simulink model "sim_tvt_2025_pos_ctrl"  (R2020a)
settings: Solver=ode4  StartTime=0.0  StopTime=30.0  FixedStep=0.01  RelTol=1e-3
values from neighbouring files (symbols this model uses):
  alfa = 0.02    [init_tvt_2025_pos_ctrl.m]
  alfa_theta = 20    [init_tvt_2025_pos_ctrl.m]
  alfa_theta_obs = 100    [init_tvt_2025_pos_ctrl.m]
  c0 = 0.1    [init_tvt_2025_pos_ctrl.m]
  c1_diff_sigma_bar_v = diag([25; 30; 20])    [init_tvt_2025_pos_ctrl.m]
  c1v = diag([5.8; 6.5; 6.5])    [init_tvt_2025_pos_ctrl.m]
  c2_diff_sigma_bar_v = diag([50; 50; 10])    [init_tvt_2025_pos_ctrl.m]
  c2v = diag([5.8; 6.5; 6.5])    [init_tvt_2025_pos_ctrl.m]
  c3_diff_sigma_bar_v = diag([15; 15; 10])    [init_tvt_2025_pos_ctrl.m]
  c3v = diag([4.8; 6.4; 6.0])    [init_tvt_2025_pos_ctrl.m]
  delta_p_i_0 = zeros(3, NF)    [init_tvt_2025_pos_ctrl.m]
  delta_v_i_0 = zeros(3, NF)    [init_tvt_2025_pos_ctrl.m]
  dp_aa_t = 0.2 * ones(3, 5) + ( 1.0 - 0.2 ) * rand(3, 5)    [init_tvt_2025_pos_ctrl.m]
  dp_ff_t = [ 0.4 * ones(1, 5) + ( 1.0 - 0.4 ) * rand(1, 5);                      0.4 * ones(1, 5) + ( 1.0 - 0.4 ) * rand(1, 5);                      0.2 * ones(1, 5) + ( 0.6 - 0.2 ) * rand(1, 5) ]    [init_tvt_2025_pos_ctrl.m]
  dp_phi_t = ( - pi / 2 ) * ones(3, 5) + ( pi / 2 - ( - pi / 2 ) ) * rand(3, 5)    [init_tvt_2025_pos_ctrl.m]
  eps0 = [0.05; 0.01; 0.01]    [init_tvt_2025_pos_ctrl.m]
  eta_ld_hat_init = zeros(3,NF)    [init_tvt_2025_pos_ctrl.m]
  etai_0 = zeros(3,5)    [init_tvt_2025_pos_ctrl.m]
  gamma0 = diag([1, 1, 1])    [init_tvt_2025_pos_ctrl.m]
  k_phi = diag([10, 10, 10])    [init_tvt_2025_pos_ctrl.m]
  k_theta = diag([5, 5, 5])    [init_tvt_2025_pos_ctrl.m]
  kai0 = [15; 10; 10]    [init_tvt_2025_pos_ctrl.m]
  kai_1_t = 0.02    [init_tvt_2025_pos_ctrl.m]
  kai_3_t = 0.1    [init_tvt_2025_pos_ctrl.m]
  ksi_ld_hat_init = zeros(3,NF)    [init_tvt_2025_pos_ctrl.m]
  ksii_0 = zeros(3,5)    [init_tvt_2025_pos_ctrl.m]
  l1v = diag([20; 20; 20])    [init_tvt_2025_pos_ctrl.m]
  l2v = diag([30; 30; 30])    [init_tvt_2025_pos_ctrl.m]
  lam0 = [15; 10; 10]    [init_tvt_2025_pos_ctrl.m]
  lam1 = diag([5,5,5])    [init_tvt_2025_pos_ctrl.m]
  lam2 = diag([5,5,5])    [init_tvt_2025_pos_ctrl.m]
  lam3 = diag([5,5,5])    [init_tvt_2025_pos_ctrl.m]
  lam4 = diag([5,5,5])    [init_tvt_2025_pos_ctrl.m]
  Lamd_diff_sigma_bar_v = 0.5    [init_tvt_2025_pos_ctrl.m]
  mass_i = zeros(1,NF)    [init_tvt_2025_pos_ctrl.m]
  Mii = diag([1;0;0;0;1])    [init_tvt_2025_pos_ctrl.m]
  pos0 = zeros(3, 1)    [init_tvt_2025_pos_ctrl.m]
  pos_bar_init = zeros(3,NF)    [init_tvt_2025_pos_ctrl.m]
  PZ0 = P0(3)    [init_tvt_2025_pos_ctrl.m]
  PZ1 = 10    [init_tvt_2025_pos_ctrl.m]
  Qci_init = repmat([1;0;0;0],1,NF)    [init_tvt_2025_pos_ctrl.m]
  R0 = 4    [init_tvt_2025_pos_ctrl.m]
  R1 = 8    [init_tvt_2025_pos_ctrl.m]
  Rx2 = 10    [init_tvt_2025_pos_ctrl.m]
  Ry2 = 6    [init_tvt_2025_pos_ctrl.m]
  Rz2 = 4    [init_tvt_2025_pos_ctrl.m]
  T0 = 0    [init_tvt_2025_pos_ctrl.m]
  T1 = tseq1    (= 10)    [init_tvt_2025_pos_ctrl.m]
  T12 = tseq1 + tseq12    (= 20)    [init_tvt_2025_pos_ctrl.m]
  T2 = tseq1 + tseq12 + tseq2    (= 30)    [init_tvt_2025_pos_ctrl.m]
  theta0 = ( 2 / 5 ) * pi    (= 1.25663706144)    [init_tvt_2025_pos_ctrl.m]
  vel0 = zeros(3, 1)    [init_tvt_2025_pos_ctrl.m]
  vel_bar_init = zeros(3,NF)    [init_tvt_2025_pos_ctrl.m]
  Wij = [0,0,1,0,0;              0,0,1,1,0;              1,0,0,0,1;              0,1,1,0,0;              0,0,1,0,0]    [init_tvt_2025_pos_ctrl.m]
  X1 = 8    [init_tvt_2025_pos_ctrl.m]
  X2 = 2    [init_tvt_2025_pos_ctrl.m]
  X3 = 3    [init_tvt_2025_pos_ctrl.m]
  Y1 = 10    [init_tvt_2025_pos_ctrl.m]
  Y2 = 2    [init_tvt_2025_pos_ctrl.m]
  Y3 = 4    [init_tvt_2025_pos_ctrl.m]
  Z1 = 4    [init_tvt_2025_pos_ctrl.m]
  Z2 = -6    [init_tvt_2025_pos_ctrl.m]
  Z3 = 2    [init_tvt_2025_pos_ctrl.m]
  zeta_diff_sigma_bar_v = 0.08    [init_tvt_2025_pos_ctrl.m]
undefined symbols (not defined in the file or in its folder): cal_frac_squ, p_alfav1, p_alfav2, p_gamma1_pos, p_gamma1_vel, p_gamma2_pos, p_gamma2_vel, q_alfav1, q_alfav2, q_gamma1_pos, q_gamma1_vel, q_gamma2_pos, q_gamma2_vel
(part 1 of 5)
settings Model: Creator=zzy  LastModifiedBy=Hershey.A
settings DataIOCC: ReturnWorkspaceOutputs=off
settings DebuggingCC: ArithmeticOperatorsInVariantConditions=warning
settings SFSimCC: SimUseLocalCustomCode=off  CustomCodeUndefinedFunction=UseInterfaceOnly
settings RTWCC: RTWUseLocalCustomCode=off

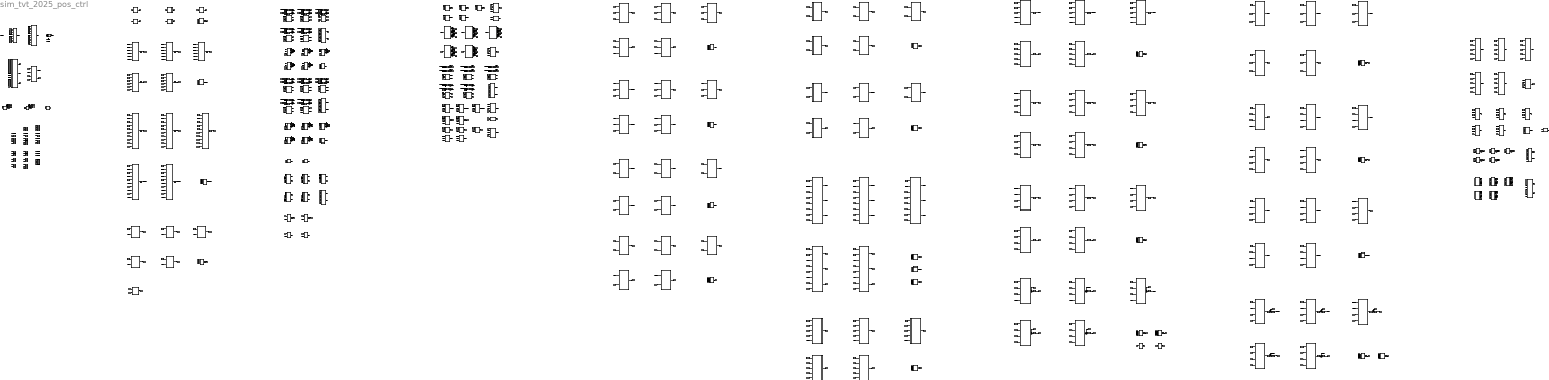
== system sim_tvt_2025_pos_ctrl ==
  Add{,1..9} (10 alike) : Sum
  Clock : Clock
  Constant{,3,6,9,14,17,22,27,32,37} (10 alike) : Constant  Value=eps0
  Constant{1,4,7,10,12,18,23,28,33,38,61,63,65,67,69,71,73,75,77,79,223,227,232,236,240} (25 alike) : Constant  Value=Wij
  Constant{100,102,107,112,117} (5 alike) : Constant  Value=p_alfav1
  Constant{101,103,108,113,118} (5 alike) : Constant  Value=alfa_theta
  Constant{97,104,109,114,119} (5 alike) : Constant  Value=q_alfav1
  Constant{98,105,110,115,120} (5 alike) : Constant  Value=p_alfav2
  Constant{99,106,111,116,121} (5 alike) : Constant  Value=q_alfav2
  Constant{2,5,8,11,13,19,24,29,34,39,224,228,233,237,242} (15 alike) : Constant  Value=Mii
  Constant{122,124,126,128,140} (5 alike) : Constant  Value=c1v
  Constant{123,125,127,139,141} (5 alike) : Constant  Value=c2v
  Constant{47..49,129..132,198,283..284} (10 alike) : Constant  Value=alfa_theta_obs
  Constant{62,68,133,200,203,206,210,213,230,263} (10 alike) : Constant  Value=l1v
  Constant{92..96,142..146} (10 alike) : Constant  Value=c3v
  Constant{91,147..150} (5 alike) : Constant  Value=lam1
  Constant{15,20,25,30,35} (5 alike) : Constant  Value=kai0
  Constant{151..160} (10 alike) : Constant  Value=gamma0
  Constant{16,21,26,31,36,40..44} (10 alike) : Constant  Value=lam0
  Constant161 : Constant  Value=T1
  Constant{162..166} (5 alike) : Constant  Value=k_theta
  Constant{167..176} (10 alike) : Constant  Value=k_phi
  Constant177 : Constant  Value=R0
  Constant178 : Constant  Value=R1
  Constant179 : Constant  Value=T0
  Constant180 : Constant  Value=Rz2
  Constant181 : Constant  Value=Ry2
  Constant182 : Constant  Value=Rx2
  Constant183 : Constant  Value=X1
  Constant184 : Constant  Value=X2
  Constant185 : Constant  Value=Y1
  Constant186 : Constant  Value=Y2
  Constant187 : Constant  Value=T2
  Constant188 : Constant  Value=R0
  Constant189 : Constant  Value=R1
  Constant190 : Constant  Value=Rx2
  Constant191 : Constant  Value=mass_i
  Constant192 : Constant  Value=Ry2
  Constant193 : Constant  Value=Rz2
  Constant194 : Constant  Value=T2
  Constant195 : Constant  Value=T1
  Constant196 : Constant  Value=PZ0
  Constant197 : Constant  Value=PZ1
  Constant{45..46,66,199,202,205,209,212,219,252} (10 alike) : Constant  Value=l2v
  Constant201 : Constant  Value=delta_v_i_0(:,1)
  Constant204 : Constant  Value=delta_v_i_0(:,2)
  Constant207 : Constant  Value=delta_v_i_0(:,3)
  Constant208 : Constant  Value=delta_p_i_0(:,1)
  Constant211 : Constant  Value=delta_v_i_0(:,4)
  Constant214 : Constant  Value=delta_v_i_0(:,5)
  Constant{215,220,270,275,279} (5 alike) : Constant  Value=p_gamma1_pos
  Constant{216,267,271,276,280} (5 alike) : Constant  Value=q_gamma1_pos
  Constant{217,268,272,277,281} (5 alike) : Constant  Value=p_gamma2_pos
  Constant{218,269,273,278,282} (5 alike) : Constant  Value=q_gamma2_pos
  Constant221 : Constant  Value=Z1
  Constant222 : Constant  Value=Z2
  Constant225 : Constant  Value=theta0
  Constant226 : Constant  Value=Z3
  Constant229 : Constant  Value=Y3
  Constant231 : Constant  Value=kai_1_t
  Constant234 : Constant  Value=X3
  Constant235 : Constant  Value=kai_3_t
  Constant238 : Constant  Value=T1
  Constant239 : Constant  Value=T12
  Constant241 : Constant  Value=delta_p_i_0(:,2)
  Constant{243,286,289,292,295} (5 alike) : Constant  Value=dp_phi_t
  Constant{244,287,290,293,296} (5 alike) : Constant  Value=dp_ff_t
  Constant{245,249,254,258,262} (5 alike) : Constant  Value=p_gamma1_vel
  Constant{246,250,255,259,264} (5 alike) : Constant  Value=q_gamma1_vel
  Constant{247,251,256,260,265} (5 alike) : Constant  Value=p_gamma2_vel
  Constant{248,253,257,261,266} (5 alike) : Constant  Value=q_gamma2_vel
  Constant274 : Constant  Value=delta_p_i_0(:,3)
  Constant{285,288,291,294,297} (5 alike) : Constant  Value=dp_aa_t
  Constant{50,53,55,57,59} (5 alike) : Constant  Value=c0
  Constant51 : Constant  Value=Qci_init
  Constant{52,54,56,58,60} (5 alike) : Constant  Value=alfa
  Constant64 : Constant  Value=delta_p_i_0(:,4)
  Constant70 : Constant  Value=delta_p_i_0(:,5)
  Constant{72,74,76,78,80} (5 alike) : Constant  Value=lam4
  Constant{81..85} (5 alike) : Constant  Value=lam3
  Constant{86..90} (5 alike) : Constant  Value=lam2
  Demux{1..10,12,22..32,68..80,88,92..97} (42 alike) : Demux  Outputs=3
  Display{6,12..25,35..59,64..68,76..95} (65 alike) : Display
  Interpreted MATLAB Function{20..29,41..60} (30 alike) : MATLABFcn  MATLABFcn=cal_frac_squ(u(1:3),u(4),u(5))
  Memory : Memory  InitialCondition=repmat(eye(3),1,1,5)
  Memory1 : Memory  InitialCondition=etai_0
  Memory10 : Memory  InitialCondition=pos_bar_init
  Memory11 : Memory  InitialCondition=ksi_ld_hat_init
  Memory{5..6,12..15,17,19..22} (11 alike) : Memory  InitialCondition=zeros(3,5)
  Memory16 : Memory  InitialCondition=pos_bar_init
  Memory18 : Memory  InitialCondition=vel_bar_init
  Memory2 : Memory  InitialCondition=ksii_0
  Memory23 : Memory  InitialCondition=vel_bar_init
  Memory3 : Memory  InitialCondition=eta_ld_hat_init
  Memory4 : Memory  InitialCondition=zeros(1,5)
  Memory7 : Memory  InitialCondition=ksi_ld_hat_init
  Memory8 : Memory  InitialCondition=pos_bar_init
  Memory9 : Memory  InitialCondition=zeros(1,5)
  Mux{86..108,119,130..135} (30 alike) : Mux  Inputs=2
  Mux{19..28,109..118,120..129} (30 alike) : Mux  Inputs=3
  Phi_sec_sigma_i agent 1 : MATLAB Function  TreatAsAtomicUnit=on
  Phi_sec_sigma_i agent 2 : MATLAB Function  TreatAsAtomicUnit=on
  Phi_sec_sigma_i agent 3 : MATLAB Function  TreatAsAtomicUnit=on
  Phi_sec_sigma_i agent 4 : MATLAB Function  TreatAsAtomicUnit=on
  Phi_sec_sigma_i agent 5 : MATLAB Function  TreatAsAtomicUnit=on
  Step : Step  Time=T1+0.01  SampleTime=0
  To Workspace : ToWorkspace  VariableName=beta_i  SampleTime=-1
  To Workspace1 : ToWorkspace  VariableName=dp_hat_vec  SampleTime=-1
  To Workspace10 : ToWorkspace  VariableName=eta_ld_hat  SampleTime=-1
  To Workspace11 : ToWorkspace  VariableName=sigma_bar_v_hat_vec  SampleTime=-1
  To Workspace12 : ToWorkspace  VariableName=sigma_bar_v_vec  SampleTime=-1
  To Workspace13 : ToWorkspace  VariableName=sigma_bar_v_tilt_vec  SampleTime=-1
  To Workspace14 : ToWorkspace  VariableName=ui  SampleTime=-1
  To Workspace15 : ToWorkspace  VariableName=rho_err  SampleTime=-1
  To Workspace16 : ToWorkspace  VariableName=pos_bar  SampleTime=-1
  To Workspace17 : ToWorkspace  VariableName=rho_hat  SampleTime=-1
  To Workspace18 : ToWorkspace  VariableName=tk_trig  SampleTime=-1
  To Workspace19 : ToWorkspace  VariableName=sigma_v_vec  SampleTime=-1
  To Workspace2 : ToWorkspace  VariableName=dp_vec  SampleTime=-1
  To Workspace20 : ToWorkspace  VariableName=d_beta_i  SampleTime=-1
  To Workspace21 : ToWorkspace  VariableName=err_vel  SampleTime=-1
  To Workspace22 : ToWorkspace  VariableName=err_pos  SampleTime=-1
  To Workspace23 : ToWorkspace  VariableName=yi  SampleTime=-1
  To Workspace24 : ToWorkspace  VariableName=vel_bar  SampleTime=-1
  To Workspace25 : ToWorkspace  VariableName=d_yi  SampleTime=-1
  To Workspace26 : ToWorkspace  VariableName=err_pos_bar  SampleTime=-1
  To Workspace27 : ToWorkspace  VariableName=err_vel_bar  SampleTime=-1
  To Workspace28 : ToWorkspace  VariableName=theta_i  SampleTime=-1
  To Workspace29 : ToWorkspace  VariableName=ksi_ld_hat_tk  SampleTime=-1
  To Workspace3 : ToWorkspace  VariableName=u0  SampleTime=-1
  To Workspace30 : ToWorkspace  VariableName=pos_bar_tk  SampleTime=-1
  To Workspace31 : ToWorkspace  VariableName=phi  SampleTime=-1
  To Workspace32 : ToWorkspace  VariableName=d_phi  SampleTime=-1
  To Workspace33 : ToWorkspace  VariableName=ksi_track_err_vec  SampleTime=-1
  To Workspace34 : ToWorkspace  VariableName=eta_track_err_vec  SampleTime=-1
  To Workspace35 : ToWorkspace  VariableName=delta_ksi_vec  SampleTime=-1
  To Workspace36 : ToWorkspace  VariableName=delta_eta_vec  SampleTime=-1
  To Workspace37 : ToWorkspace  VariableName=eta_d_est_vec  SampleTime=-1
  To Workspace38 : ToWorkspace  VariableName=ksi_est_err  SampleTime=-1
  To Workspace39 : ToWorkspace  VariableName=ksi_d_est_vec  SampleTime=-1
  To Workspace4 : ToWorkspace  VariableName=eta0  SampleTime=-1
  To Workspace40 : ToWorkspace  VariableName=eta_est_err  SampleTime=-1
  To Workspace41 : ToWorkspace  VariableName=eta_ld_est_err  SampleTime=-1
  To Workspace42 : ToWorkspace  VariableName=ksi_ld_est_err  SampleTime=-1
  To Workspace5 : ToWorkspace  VariableName=ksi0  SampleTime=-1
  To Workspace6 : ToWorkspace  VariableName=dp_tilt_vec  SampleTime=-1
  To Workspace7 : ToWorkspace  VariableName=eta_i_vec  SampleTime=-1
  To Workspace8 : ToWorkspace  VariableName=ksi_i_vec  SampleTime=-1
  To Workspace9 : ToWorkspace  VariableName=ksi_ld_hat  SampleTime=-1
  beta_hat Integrator {1..5} (5 alike) : Integrator
  cal Di agent 1 : MATLAB Function  TreatAsAtomicUnit=on
  cal Di agent 2 : MATLAB Function  TreatAsAtomicUnit=on
  cal Di agent 3 : MATLAB Function  TreatAsAtomicUnit=on
  cal Di agent 4 : MATLAB Function  TreatAsAtomicUnit=on
  cal Di agent 5 : MATLAB Function  TreatAsAtomicUnit=on
  cal Rci from ui : MATLAB Function  TreatAsAtomicUnit=on
  cal Rei : MATLAB Function  TreatAsAtomicUnit=on
  cal Ri : MATLAB Function  TreatAsAtomicUnit=on
  cal abs 21 : MATLAB Function  TreatAsAtomicUnit=on
  cal abs 22 : MATLAB Function  TreatAsAtomicUnit=on
  cal abs 23 : MATLAB Function  TreatAsAtomicUnit=on
  cal abs 24 : MATLAB Function  TreatAsAtomicUnit=on
  cal abs 25 : MATLAB Function  TreatAsAtomicUnit=on
  cal abs 26 : MATLAB Function  TreatAsAtomicUnit=on
  cal abs 27 : MATLAB Function  TreatAsAtomicUnit=on
  cal abs 28 : MATLAB Function  TreatAsAtomicUnit=on
  cal abs 29 : MATLAB Function  TreatAsAtomicUnit=on
  cal abs 30 : MATLAB Function  TreatAsAtomicUnit=on
  cal abs 41 : MATLAB Function  TreatAsAtomicUnit=on
  cal abs 42 : MATLAB Function  TreatAsAtomicUnit=on
  cal abs 43 : MATLAB Function  TreatAsAtomicUnit=on
  cal abs 44 : MATLAB Function  TreatAsAtomicUnit=on
  cal abs 45 : MATLAB Function  TreatAsAtomicUnit=on
  cal abs 46 : MATLAB Function  TreatAsAtomicUnit=on
  cal abs 47 : MATLAB Function  TreatAsAtomicUnit=on
  cal abs 48 : MATLAB Function  TreatAsAtomicUnit=on
  cal abs 49 : MATLAB Function  TreatAsAtomicUnit=on
  cal abs 50 : MATLAB Function  TreatAsAtomicUnit=on
  cal abs 51 : MATLAB Function  TreatAsAtomicUnit=on
  cal abs 52 : MATLAB Function  TreatAsAtomicUnit=on
  cal abs 53 : MATLAB Function  TreatAsAtomicUnit=on
  cal abs 54 : MATLAB Function  TreatAsAtomicUnit=on
  cal abs 55 : MATLAB Function  TreatAsAtomicUnit=on
  cal abs 56 : MATLAB Function  TreatAsAtomicUnit=on
  cal abs 57 : MATLAB Function  TreatAsAtomicUnit=on
  cal abs 58 : MATLAB Function  TreatAsAtomicUnit=on
  cal abs 59 : MATLAB Function  TreatAsAtomicUnit=on
  cal abs 60 : MATLAB Function  TreatAsAtomicUnit=on
  cal betai agent 1 : MATLAB Function  TreatAsAtomicUnit=on
  cal betai agent 2 : MATLAB Function  TreatAsAtomicUnit=on
  cal betai agent 3 : MATLAB Function  TreatAsAtomicUnit=on
  cal betai agent 4 : MATLAB Function  TreatAsAtomicUnit=on
  cal betai agent 5 : MATLAB Function  TreatAsAtomicUnit=on
  cal combine sigma_bar_v : MATLAB Function  TreatAsAtomicUnit=on
  cal combine sigma_bar_v_tilt : MATLAB Function  TreatAsAtomicUnit=on
  cal d_betai agent 1 : MATLAB Function  TreatAsAtomicUnit=on
  cal d_betai agent 2 : MATLAB Function  TreatAsAtomicUnit=on
  cal d_betai agent 3 : MATLAB Function  TreatAsAtomicUnit=on
  cal d_betai agent 4 : MATLAB Function  TreatAsAtomicUnit=on
  cal d_betai agent 5 : MATLAB Function  TreatAsAtomicUnit=on
  cal d_yi : MATLAB Function  TreatAsAtomicUnit=on
  cal differentiator d_sigma_bar_v_hat agent 1 : Subsystem
  cal differentiator d_sigma_bar_v_hat agent 2 : Subsystem
  cal differentiator d_sigma_bar_v_hat agent 3 : Subsystem
  cal differentiator d_sigma_bar_v_hat agent 4 : Subsystem
  cal differentiator d_sigma_bar_v_hat agent 5 : Subsystem
  cal disturbance observation error dp_tilt : MATLAB Function  TreatAsAtomicUnit=on
  cal dp_hat agent 1 : MATLAB Function  TreatAsAtomicUnit=on
  cal dp_hat agent 2 : MATLAB Function  TreatAsAtomicUnit=on
  cal dp_hat agent 3 : MATLAB Function  TreatAsAtomicUnit=on
  cal dp_hat agent 4 : MATLAB Function  TreatAsAtomicUnit=on
  cal dp_hat agent 5 : MATLAB Function  TreatAsAtomicUnit=on
  cal err_pos_bar_i agent 1 : MATLAB Function  TreatAsAtomicUnit=on
  cal err_pos_bar_i agent 2 : MATLAB Function  TreatAsAtomicUnit=on
  cal err_pos_bar_i agent 3 : MATLAB Function  TreatAsAtomicUnit=on
  cal err_pos_bar_i agent 4 : MATLAB Function  TreatAsAtomicUnit=on
  cal err_pos_bar_i agent 5 : MATLAB Function  TreatAsAtomicUnit=on
  cal err_pos_i agent 1 : MATLAB Function  TreatAsAtomicUnit=on
  cal err_pos_i agent 2 : MATLAB Function  TreatAsAtomicUnit=on
  cal err_pos_i agent 3 : MATLAB Function  TreatAsAtomicUnit=on
  cal err_pos_i agent 4 : MATLAB Function  TreatAsAtomicUnit=on
  cal err_pos_i agent 5 : MATLAB Function  TreatAsAtomicUnit=on
  cal err_vel_bar_i agent 1 : MATLAB Function  TreatAsAtomicUnit=on
  cal err_vel_bar_i agent 2 : MATLAB Function  TreatAsAtomicUnit=on
  cal err_vel_bar_i agent 3 : MATLAB Function  TreatAsAtomicUnit=on
  cal err_vel_bar_i agent 4 : MATLAB Function  TreatAsAtomicUnit=on
  cal err_vel_bar_i agent 5 : MATLAB Function  TreatAsAtomicUnit=on
  cal err_vel_i agent 1 : MATLAB Function  TreatAsAtomicUnit=on
  cal err_vel_i agent 2 : MATLAB Function  TreatAsAtomicUnit=on
  cal err_vel_i agent 3 : MATLAB Function  TreatAsAtomicUnit=on
  cal err_vel_i agent 4 : MATLAB Function  TreatAsAtomicUnit=on
  cal err_vel_i agent 5 : MATLAB Function  TreatAsAtomicUnit=on
  cal follower desire position estimate error : MATLAB Function  TreatAsAtomicUnit=on
  cal follower desire velocity estimate error : MATLAB Function  TreatAsAtomicUnit=on
  cal leader position estimate error : MATLAB Function  TreatAsAtomicUnit=on
  cal leader position observation : MATLAB Function  TreatAsAtomicUnit=on
  cal leader velocity estimate error : MATLAB Function  TreatAsAtomicUnit=on
  cal leader velocity observation : MATLAB Function  TreatAsAtomicUnit=on
  cal lumped observation error agent 1 : MATLAB Function  TreatAsAtomicUnit=on
  cal lumped observation error agent 2 : MATLAB Function  TreatAsAtomicUnit=on
  cal lumped observation error agent 3 : MATLAB Function  TreatAsAtomicUnit=on
  cal lumped observation error agent 4 : MATLAB Function  TreatAsAtomicUnit=on
  cal lumped observation error agent 5 : MATLAB Function  TreatAsAtomicUnit=on
  cal phi agent 1 : MATLAB Function  TreatAsAtomicUnit=on
  cal phi agent 2 : MATLAB Function  TreatAsAtomicUnit=on
  cal phi agent 3 : MATLAB Function  TreatAsAtomicUnit=on
  cal phi agent 4 : MATLAB Function  TreatAsAtomicUnit=on
  cal phi agent 5 : MATLAB Function  TreatAsAtomicUnit=on
  cal pos_bar_i agent 1 : MATLAB Function  TreatAsAtomicUnit=on
  cal pos_bar_i agent 2 : MATLAB Function  TreatAsAtomicUnit=on
  cal pos_bar_i agent 3 : MATLAB Function  TreatAsAtomicUnit=on
  cal pos_bar_i agent 4 : MATLAB Function  TreatAsAtomicUnit=on
  cal pos_bar_i agent 5 : MATLAB Function  TreatAsAtomicUnit=on
  cal rho_err_vec : MATLAB Function  TreatAsAtomicUnit=on
  cal sigma_bar_v_hat agent 1 : MATLAB Function  TreatAsAtomicUnit=on
  cal sigma_bar_v_hat agent 2 : MATLAB Function  TreatAsAtomicUnit=on
  cal sigma_bar_v_hat agent 3 : MATLAB Function  TreatAsAtomicUnit=on
  cal sigma_bar_v_hat agent 4 : MATLAB Function  TreatAsAtomicUnit=on
  cal sigma_bar_v_hat agent 5 : MATLAB Function  TreatAsAtomicUnit=on
  cal theta_eta_est_err_tilt agent 1 : MATLAB Function  TreatAsAtomicUnit=on
  cal theta_eta_est_err_tilt agent 2 : MATLAB Function  TreatAsAtomicUnit=on
  cal theta_eta_est_err_tilt agent 3 : MATLAB Function  TreatAsAtomicUnit=on
  cal theta_eta_est_err_tilt agent 4 : MATLAB Function  TreatAsAtomicUnit=on
  cal theta_eta_est_err_tilt agent 5 : MATLAB Function  TreatAsAtomicUnit=on
  cal theta_ksi_est_err_tilt agent 1 : MATLAB Function  TreatAsAtomicUnit=on
  cal theta_ksi_est_err_tilt agent 2 : MATLAB Function  TreatAsAtomicUnit=on
  cal theta_ksi_est_err_tilt agent 3 : MATLAB Function  TreatAsAtomicUnit=on
  cal theta_ksi_est_err_tilt agent 4 : MATLAB Function  TreatAsAtomicUnit=on
  cal theta_ksi_est_err_tilt agent 5 : MATLAB Function  TreatAsAtomicUnit=on
  cal theta_sigma_bar_v_tilt agent 1 : MATLAB Function  TreatAsAtomicUnit=on
  cal theta_sigma_bar_v_tilt agent 2 : MATLAB Function  TreatAsAtomicUnit=on
  cal theta_sigma_bar_v_tilt agent 3 : MATLAB Function  TreatAsAtomicUnit=on
  cal theta_sigma_bar_v_tilt agent 4 : MATLAB Function  TreatAsAtomicUnit=on
  cal theta_sigma_bar_v_tilt agent 5 : MATLAB Function  TreatAsAtomicUnit=on
  cal thetai agent 1 : MATLAB Function  TreatAsAtomicUnit=on
  cal thetai agent 2 : MATLAB Function  TreatAsAtomicUnit=on
  cal thetai agent 3 : MATLAB Function  TreatAsAtomicUnit=on
  cal thetai agent 4 : MATLAB Function  TreatAsAtomicUnit=on
  cal thetai agent 5 : MATLAB Function  TreatAsAtomicUnit=on
  cal ui agent 1 : MATLAB Function  TreatAsAtomicUnit=on
  cal ui agent 2 : MATLAB Function  TreatAsAtomicUnit=on
  cal ui agent 3 : MATLAB Function  TreatAsAtomicUnit=on
  cal ui agent 4 : MATLAB Function  TreatAsAtomicUnit=on
  cal ui agent 5 : MATLAB Function  TreatAsAtomicUnit=on
  cal vel_bar_i agent 1 : MATLAB Function  TreatAsAtomicUnit=on
  cal vel_bar_i agent 2 : MATLAB Function  TreatAsAtomicUnit=on
  cal vel_bar_i agent 3 : MATLAB Function  TreatAsAtomicUnit=on
  cal vel_bar_i agent 4 : MATLAB Function  TreatAsAtomicUnit=on
  cal vel_bar_i agent 5 : MATLAB Function  TreatAsAtomicUnit=on
  cal virtual control sigma_v agent 1 : MATLAB Function  TreatAsAtomicUnit=on
  cal virtual control sigma_v agent 2 : MATLAB Function  TreatAsAtomicUnit=on
  cal virtual control sigma_v agent 3 : MATLAB Function  TreatAsAtomicUnit=on
  cal virtual control sigma_v agent 4 : MATLAB Function  TreatAsAtomicUnit=on
  cal virtual control sigma_v agent 5 : MATLAB Function  TreatAsAtomicUnit=on
  cal x1i agent 1 : MATLAB Function  TreatAsAtomicUnit=on
  cal x1i agent 2 : MATLAB Function  TreatAsAtomicUnit=on
  cal x1i agent 3 : MATLAB Function  TreatAsAtomicUnit=on
  cal x1i agent 4 : MATLAB Function  TreatAsAtomicUnit=on
  cal x1i agent 5 : MATLAB Function  TreatAsAtomicUnit=on
  cal x2i agent 1 : MATLAB Function  TreatAsAtomicUnit=on
  cal x2i agent 2 : MATLAB Function  TreatAsAtomicUnit=on
  cal x2i agent 3 : MATLAB Function  TreatAsAtomicUnit=on
  cal x2i agent 4 : MATLAB Function  TreatAsAtomicUnit=on
  cal x2i agent 5 : MATLAB Function  TreatAsAtomicUnit=on
  cal x3i agent 1 : MATLAB Function  TreatAsAtomicUnit=on
  cal x3i agent 2 : MATLAB Function  TreatAsAtomicUnit=on
  cal x3i agent 3 : MATLAB Function  TreatAsAtomicUnit=on
  cal x3i agent 4 : MATLAB Function  TreatAsAtomicUnit=on
  cal x3i agent 5 : MATLAB Function  TreatAsAtomicUnit=on
  cal x4i agent 1 : MATLAB Function  TreatAsAtomicUnit=on
  cal x4i agent 2 : MATLAB Function  TreatAsAtomicUnit=on
  cal x4i agent 3 : MATLAB Function  TreatAsAtomicUnit=on
  cal x4i agent 4 : MATLAB Function  TreatAsAtomicUnit=on
  cal x4i agent 5 : MATLAB Function  TreatAsAtomicUnit=on
  cal yi : MATLAB Function  TreatAsAtomicUnit=on
  choose eta_est_err_tilt 1 : MATLAB Function  TreatAsAtomicUnit=on
  choose eta_est_err_tilt 10 : MATLAB Function  TreatAsAtomicUnit=on
  choose eta_est_err_tilt 11 : MATLAB Function  TreatAsAtomicUnit=on
  choose eta_est_err_tilt 12 : MATLAB Function  TreatAsAtomicUnit=on
  choose eta_est_err_tilt 13 : MATLAB Function  TreatAsAtomicUnit=on
  choose eta_est_err_tilt 14 : MATLAB Function  TreatAsAtomicUnit=on
  choose eta_est_err_tilt 15 : MATLAB Function  TreatAsAtomicUnit=on
  choose eta_est_err_tilt 16 : MATLAB Function  TreatAsAtomicUnit=on
  choose eta_est_err_tilt 17 : MATLAB Function  TreatAsAtomicUnit=on
  choose eta_est_err_tilt 18 : MATLAB Function  TreatAsAtomicUnit=on
  choose eta_est_err_tilt 19 : MATLAB Function  TreatAsAtomicUnit=on
  choose eta_est_err_tilt 2 : MATLAB Function  TreatAsAtomicUnit=on
  choose eta_est_err_tilt 20 : MATLAB Function  TreatAsAtomicUnit=on
  choose eta_est_err_tilt 3 : MATLAB Function  TreatAsAtomicUnit=on
  choose eta_est_err_tilt 4 : MATLAB Function  TreatAsAtomicUnit=on
  choose eta_est_err_tilt 5 : MATLAB Function  TreatAsAtomicUnit=on
  choose eta_est_err_tilt 6 : MATLAB Function  TreatAsAtomicUnit=on
  choose eta_est_err_tilt 7 : MATLAB Function  TreatAsAtomicUnit=on
  choose eta_est_err_tilt 8 : MATLAB Function  TreatAsAtomicUnit=on
  choose eta_est_err_tilt 9 : MATLAB Function  TreatAsAtomicUnit=on
  choose ksi_est_err 21 : MATLAB Function  TreatAsAtomicUnit=on
  choose ksi_est_err 22 : MATLAB Function  TreatAsAtomicUnit=on
  choose ksi_est_err 23 : MATLAB Function  TreatAsAtomicUnit=on
  choose ksi_est_err 24 : MATLAB Function  TreatAsAtomicUnit=on
  choose ksi_est_err 25 : MATLAB Function  TreatAsAtomicUnit=on
  choose ksi_est_err 26 : MATLAB Function  TreatAsAtomicUnit=on
  choose ksi_est_err 27 : MATLAB Function  TreatAsAtomicUnit=on
  choose ksi_est_err 28 : MATLAB Function  TreatAsAtomicUnit=on
  choose ksi_est_err 29 : MATLAB Function  TreatAsAtomicUnit=on
  choose ksi_est_err 30 : MATLAB Function  TreatAsAtomicUnit=on
  combine Di_vec : MATLAB Function  TreatAsAtomicUnit=on
  combine Phi_sec_sigma_i : MATLAB Function  TreatAsAtomicUnit=on
  combine beta : MATLAB Function  TreatAsAtomicUnit=on
  combine beta_hat : MATLAB Function  TreatAsAtomicUnit=on
  combine betai1 : MATLAB Function  TreatAsAtomicUnit=on
  combine d_betai : MATLAB Function  TreatAsAtomicUnit=on
  combine d_phi : MATLAB Function  TreatAsAtomicUnit=on
  combine d_sigma_bar_v_est : MATLAB Function  TreatAsAtomicUnit=on
  combine d_xi1 : MATLAB Function  TreatAsAtomicUnit=on
  combine dp_hat : MATLAB Function  TreatAsAtomicUnit=on
  combine err_pos_bar_i : MATLAB Function  TreatAsAtomicUnit=on
  combine err_pos_i : MATLAB Function  TreatAsAtomicUnit=on
  combine err_vel_bar : MATLAB Function  TreatAsAtomicUnit=on
  combine err_vel_i : MATLAB Function  TreatAsAtomicUnit=on
  combine event trigger ksi_ld_hat_tk : MATLAB Function  TreatAsAtomicUnit=on
  combine event trigger pos_bar_tk : MATLAB Function  TreatAsAtomicUnit=on
  combine event trigger tk : MATLAB Function  TreatAsAtomicUnit=on
  combine follower desire velocity estimaters : MATLAB Function  TreatAsAtomicUnit=on
  combine follower eta ksi : MATLAB Function  TreatAsAtomicUnit=on
  combine formation control input : MATLAB Function  TreatAsAtomicUnit=on
  combine leader position estimaters : MATLAB Function  TreatAsAtomicUnit=on
  "combine lumped follower observation error " : MATLAB Function  TreatAsAtomicUnit=on
  combine lumped follower position observation error : MATLAB Function  TreatAsAtomicUnit=on
  combine lumped follower velocity observation error : MATLAB Function  TreatAsAtomicUnit=on
  combine phi : MATLAB Function  TreatAsAtomicUnit=on
  combine pos_bar_i : MATLAB Function  TreatAsAtomicUnit=on
  combine rho_hat : MATLAB Function  TreatAsAtomicUnit=on
  combine sigma_bar_v_hat : MATLAB Function  TreatAsAtomicUnit=on
  combine sigma_v : MATLAB Function  TreatAsAtomicUnit=on
  combine theta_sigma_bar_v_tilt : MATLAB Function  TreatAsAtomicUnit=on
  combine thetai : MATLAB Function  TreatAsAtomicUnit=on
  combine translational disturbance : MATLAB Function  TreatAsAtomicUnit=on
  combine ui : MATLAB Function  TreatAsAtomicUnit=on
  combine vel_bar_i : MATLAB Function  TreatAsAtomicUnit=on
  combine x1i : MATLAB Function  TreatAsAtomicUnit=on
  combine x2i : MATLAB Function  TreatAsAtomicUnit=on
  combine x3i : MATLAB Function  TreatAsAtomicUnit=on
  combine x4i : MATLAB Function  TreatAsAtomicUnit=on
  d2_sigma_bar_v_est_{1..5} (5 alike) : Scope  NumInputPorts=3
  d_phi Integrator agent {1..5} (5 alike) : Integrator  InitialCondition=zeros(3,1)
  d_sigma_bar_v_est_{1..5} (5 alike) : Scope  NumInputPorts=3
  depart Rc1 : MATLAB Function  TreatAsAtomicUnit=on
  depart Rc2 : MATLAB Function  TreatAsAtomicUnit=on
  depart Rc3 : MATLAB Function  TreatAsAtomicUnit=on
  depart Rc4 : MATLAB Function  TreatAsAtomicUnit=on
  depart Rc5 : MATLAB Function  TreatAsAtomicUnit=on
  depart Re1 : MATLAB Function  TreatAsAtomicUnit=on
  depart Re2 : MATLAB Function  TreatAsAtomicUnit=on
  depart Re3 : MATLAB Function  TreatAsAtomicUnit=on
  depart Re4 : MATLAB Function  TreatAsAtomicUnit=on
  depart Re5 : MATLAB Function  TreatAsAtomicUnit=on
  desire formation position and velocity : MATLAB Function  TreatAsAtomicUnit=on
  eta_0 : Scope  NumInputPorts=3
  eta_d_est_{1..5} (5 alike) : Scope  NumInputPorts=3
  eta_track_err_{1..5} (5 alike) : Scope  NumInputPorts=3
  fixed-time distributed follower desire position observer agent 1 : MATLAB Function  TreatAsAtomicUnit=on
  fixed-time distributed follower desire position observer agent 2 : MATLAB Function  TreatAsAtomicUnit=on
  fixed-time distributed follower desire position observer agent 3 : MATLAB Function  TreatAsAtomicUnit=on
  fixed-time distributed follower desire position observer agent 4 : MATLAB Function  TreatAsAtomicUnit=on
  fixed-time distributed follower desire position observer agent 5 : MATLAB Function  TreatAsAtomicUnit=on
  fixed-time distributed follower desire velocity observer agent 1 : MATLAB Function  TreatAsAtomicUnit=on
  fixed-time distributed follower desire velocity observer agent 2 : MATLAB Function  TreatAsAtomicUnit=on
  fixed-time distributed follower desire velocity observer agent 3 : MATLAB Function  TreatAsAtomicUnit=on
  fixed-time distributed follower desire velocity observer agent 4 : MATLAB Function  TreatAsAtomicUnit=on
  fixed-time distributed follower desire velocity observer agent 5 : MATLAB Function  TreatAsAtomicUnit=on
  follower etai Integrator agent 1 : Integrator  InitialCondition=etai_0(:,1)
  follower etai Integrator agent 2 : Integrator  InitialCondition=etai_0(:,2)
  follower etai Integrator agent 3 : Integrator  InitialCondition=etai_0(:,3)
  follower etai Integrator agent 4 : Integrator  InitialCondition=etai_0(:,4)
  follower etai Integrator agent 5 : Integrator  InitialCondition=etai_0(:,5)
  follower ksii Integrator agent 1 : Integrator  InitialCondition=ksii_0(:,1)
  follower ksii Integrator agent 2 : Integrator  InitialCondition=ksii_0(:,2)
  follower ksii Integrator agent 3 : Integrator  InitialCondition=ksii_0(:,3)
  follower ksii Integrator agent 4 : Integrator  InitialCondition=ksii_0(:,4)
  follower ksii Integrator agent 5 : Integrator  InitialCondition=ksii_0(:,5)
  follower tracking error agent 1 : MATLAB Function  TreatAsAtomicUnit=on
  follower tracking error agent 2 : MATLAB Function  TreatAsAtomicUnit=on
  follower tracking error agent 3 : MATLAB Function  TreatAsAtomicUnit=on
  follower tracking error agent 4 : MATLAB Function  TreatAsAtomicUnit=on
  follower tracking error agent 5 : MATLAB Function  TreatAsAtomicUnit=on
  generate translational disturbance agent 1 : MATLAB Function  TreatAsAtomicUnit=on
  generate translational disturbance agent 2 : MATLAB Function  TreatAsAtomicUnit=on
  generate translational disturbance agent 3 : MATLAB Function  TreatAsAtomicUnit=on
  generate translational disturbance agent 4 : MATLAB Function  TreatAsAtomicUnit=on
  generate translational disturbance agent 5 : MATLAB Function  TreatAsAtomicUnit=on
  ksi_0 : Scope  NumInputPorts=3
  ksi_d_est_{1..5} (5 alike) : Scope  NumInputPorts=3
  ksi_track_err_{1..5} (5 alike) : Scope  NumInputPorts=3
  leader control input : MATLAB Function  TreatAsAtomicUnit=on
  leader eta0 Integrator : Integrator  ExternalReset=rising  InitialConditionSource=external  InitialCondition=vel0
  leader ksi0 Integrator : Integrator  InitialCondition=pos0
  phi Integrator agent {1..5} (5 alike) : Integrator  InitialCondition=zeros(3,1)
  position observe Integrator {1..5} (5 alike) : Integrator  InitialCondition=zeros(3,1)
  process velocity : MATLAB Function  TreatAsAtomicUnit=on
  rho_hat agent 1 : MATLAB Function  TreatAsAtomicUnit=on
  rho_hat agent 2 : MATLAB Function  TreatAsAtomicUnit=on
  rho_hat agent 3 : MATLAB Function  TreatAsAtomicUnit=on
  rho_hat agent 4 : MATLAB Function  TreatAsAtomicUnit=on
  rho_hat agent 5 : MATLAB Function  TreatAsAtomicUnit=on
  set desire formation configuration : MATLAB Function  TreatAsAtomicUnit=on
  sigma_bar_v_hat Integrator {1..5} (5 alike) : Integrator  InitialCondition=zeros(3,1)
  sigma_v Integrator {1..5} (5 alike) : Integrator  InitialCondition=zeros(3,1)
  sigmai Integrator {1..5} (5 alike) : Integrator  InitialCondition=zeros(3,1)
  trans to column20 : MATLAB Function  TreatAsAtomicUnit=on
  trans to column21 : MATLAB Function  TreatAsAtomicUnit=on
  trans to column22 : MATLAB Function  TreatAsAtomicUnit=on
  trans to column23 : MATLAB Function  TreatAsAtomicUnit=on
  trans to column24 : MATLAB Function  TreatAsAtomicUnit=on
  trans to column25 : MATLAB Function  TreatAsAtomicUnit=on
  trans to column26 : MATLAB Function  TreatAsAtomicUnit=on
  trans to column27 : MATLAB Function  TreatAsAtomicUnit=on
  trans to column28 : MATLAB Function  TreatAsAtomicUnit=on
  trans to column29 : MATLAB Function  TreatAsAtomicUnit=on
  trans to column41 : MATLAB Function  TreatAsAtomicUnit=on
  trans to column42 : MATLAB Function  TreatAsAtomicUnit=on
  trans to column43 : MATLAB Function  TreatAsAtomicUnit=on
  trans to column44 : MATLAB Function  TreatAsAtomicUnit=on
  trans to column45 : MATLAB Function  TreatAsAtomicUnit=on
  trans to column46 : MATLAB Function  TreatAsAtomicUnit=on
  trans to column47 : MATLAB Function  TreatAsAtomicUnit=on
  trans to column48 : MATLAB Function  TreatAsAtomicUnit=on
  trans to column49 : MATLAB Function  TreatAsAtomicUnit=on
  trans to column50 : MATLAB Function  TreatAsAtomicUnit=on
  trans to column51 : MATLAB Function  TreatAsAtomicUnit=on
  trans to column52 : MATLAB Function  TreatAsAtomicUnit=on
  trans to column53 : MATLAB Function  TreatAsAtomicUnit=on
  trans to column54 : MATLAB Function  TreatAsAtomicUnit=on
  trans to column55 : MATLAB Function  TreatAsAtomicUnit=on
  trans to column56 : MATLAB Function  TreatAsAtomicUnit=on
  trans to column57 : MATLAB Function  TreatAsAtomicUnit=on
  trans to column58 : MATLAB Function  TreatAsAtomicUnit=on
  trans to column59 : MATLAB Function  TreatAsAtomicUnit=on
  trans to column60 : MATLAB Function  TreatAsAtomicUnit=on
  uav translational dynamics agent 1 : MATLAB Function  TreatAsAtomicUnit=on
  uav translational dynamics agent 2 : MATLAB Function  TreatAsAtomicUnit=on
  uav translational dynamics agent 3 : MATLAB Function  TreatAsAtomicUnit=on
  uav translational dynamics agent 4 : MATLAB Function  TreatAsAtomicUnit=on
  uav translational dynamics agent 5 : MATLAB Function  TreatAsAtomicUnit=on
  update betai agent 1 : MATLAB Function  TreatAsAtomicUnit=on
  update betai agent 2 : MATLAB Function  TreatAsAtomicUnit=on
  update betai agent 3 : MATLAB Function  TreatAsAtomicUnit=on
  update betai agent 4 : MATLAB Function  TreatAsAtomicUnit=on
  update betai agent 5 : MATLAB Function  TreatAsAtomicUnit=on
  update event trigger state agent 1 : MATLAB Function  TreatAsAtomicUnit=on
  update event trigger state agent 2 : MATLAB Function  TreatAsAtomicUnit=on
  update event trigger state agent 3 : MATLAB Function  TreatAsAtomicUnit=on
  update event trigger state agent 4 : MATLAB Function  TreatAsAtomicUnit=on
  update event trigger state agent 5 : MATLAB Function  TreatAsAtomicUnit=on
  update sigmai agent 1 : MATLAB Function  TreatAsAtomicUnit=on
  update sigmai agent 2 : MATLAB Function  TreatAsAtomicUnit=on
  update sigmai agent 3 : MATLAB Function  TreatAsAtomicUnit=on
  update sigmai agent 4 : MATLAB Function  TreatAsAtomicUnit=on
  update sigmai agent 5 : MATLAB Function  TreatAsAtomicUnit=on
  velocity observe Integrator {1..5} (5 alike) : Integrator  InitialCondition=zeros(3,1)
  x1i Integrator agent 1 : Integrator  InitialCondition=pos_bar_init(:,1)
  x1i Integrator agent 2 : Integrator  InitialCondition=pos_bar_init(:,2)
  x1i Integrator agent 3 : Integrator  InitialCondition=pos_bar_init(:,3)
  x1i Integrator agent 4 : Integrator  InitialCondition=pos_bar_init(:,4)
  x1i Integrator agent 5 : Integrator  InitialCondition=pos_bar_init(:,5)
  x2i Integrator agent {1..5} (5 alike) : Integrator  InitialCondition=zeros(3,1)
  x3i Integrator agent {1..5} (5 alike) : Integrator  InitialCondition=zeros(3,1)
  x4i Integrator agent {1..5} (5 alike) : Integrator  InitialCondition=zeros(3,1)
  wires:
  follower etai Integrator agent 1/1 -> [eta_1], follower ksii Integrator agent 1/1
  follower etai Integrator agent 2/1 -> [eta_2], follower ksii Integrator agent 2/1
  follower etai Integrator agent 3/1 -> [eta_3], follower ksii Integrator agent 3/1
  follower etai Integrator agent 4/1 -> [eta_4], follower ksii Integrator agent 4/1
  follower etai Integrator agent 5/1 -> [eta_5], follower ksii Integrator agent 5/1
  follower ksii Integrator agent 1/1 -> [ksi_1]
  follower ksii Integrator agent 2/1 -> [ksi_2]
  follower ksii Integrator agent 3/1 -> [ksi_3]
  follower ksii Integrator agent 4/1 -> [ksi_4]
  follower ksii Integrator agent 5/1 -> [ksi_5]
  [eta_1] -> combine formation control input/1(eta_1)
  [eta_2] -> combine formation control input/2(eta_2)
  [eta_3] -> combine formation control input/3(eta_3)
  [eta_4] -> combine formation control input/4(eta_4)
  [eta_5] -> combine formation control input/5(eta_5)
  [ksi_1] -> combine formation control input/6(ksi_1)
  [ksi_2] -> combine formation control input/7(ksi_2)
  [ksi_3] -> combine formation control input/8(ksi_3)
  [ksi_4] -> combine formation control input/9(ksi_4)
  [ksi_5] -> combine formation control input/10(ksi_5)
  [ksi_i_vec] -> follower tracking error agent 1/3(ksi_i_vec)
  [eta_i_vec] -> follower tracking error agent 1/4(eta_i_vec)
  [ksi0] -> follower tracking error agent 1/5(ksi0)
  [eta0] -> follower tracking error agent 1/6(eta0)
  follower tracking error agent 1/2(eta_track_err_1) -> Display13/1, Demux24/1, [eta_track_err_1]
  follower tracking error agent 1/1(ksi_track_err_1) -> Display12/1, Demux23/1, [ksi_track_err_1]
  [eta0] -> follower tracking error agent 2/6(eta0)
  [ksi0] -> follower tracking error agent 2/5(ksi0)
  [eta_i_vec] -> follower tracking error agent 2/4(eta_i_vec)
  follower tracking error agent 2/2(eta_track_err_2) -> Display15/1, Demux26/1, [eta_track_err_2]
  [ksi_i_vec] -> follower tracking error agent 2/3(ksi_i_vec)
  follower tracking error agent 2/1(ksi_track_err_2) -> Display14/1, Demux25/1, [ksi_track_err_2]
  follower tracking error agent 3/2(eta_track_err_3) -> Display17/1, Demux28/1, [eta_track_err_3]
  follower tracking error agent 3/1(ksi_track_err_3) -> Display16/1, Demux27/1, [ksi_track_err_3]
  [eta0] -> follower tracking error agent 3/6(eta0)
  [eta_i_vec] -> follower tracking error agent 3/4(eta_i_vec)
  [ksi_i_vec] -> follower tracking error agent 3/3(ksi_i_vec)
  [ksi0] -> follower tracking error agent 3/5(ksi0)
  [ksi_i_vec] -> follower tracking error agent 4/3(ksi_i_vec)
  [ksi0] -> follower tracking error agent 4/5(ksi0)
  [eta_i_vec] -> follower tracking error agent 4/4(eta_i_vec)
  [eta0] -> follower tracking error agent 4/6(eta0)
  follower tracking error agent 4/2(eta_track_err_4) -> Display19/1, Demux30/1, [eta_track_err_4]
  follower tracking error agent 4/1(ksi_track_err_4) -> Display18/1, Demux29/1, [ksi_track_err_4]
  follower tracking error agent 5/1(ksi_track_err_5) -> Display20/1, Demux31/1, [ksi_track_err_5]
  [ksi_i_vec] -> follower tracking error agent 5/3(ksi_i_vec)
  [eta0] -> follower tracking error agent 5/6(eta0)
  [ksi0] -> follower tracking error agent 5/5(ksi0)
  [eta_i_vec] -> follower tracking error agent 5/4(eta_i_vec)
  follower tracking error agent 5/2(eta_track_err_5) -> Display21/1, Demux32/1, [eta_track_err_5]
  [ksi_track_err_1] -> combine follower eta ksi/1(ksi_track_err_1)
  [ksi_track_err_2] -> combine follower eta ksi/2(ksi_track_err_2)
  [ksi_track_err_3] -> combine follower eta ksi/3(ksi_track_err_3)
  [ksi_track_err_4] -> combine follower eta ksi/4(ksi_track_err_4)
  [ksi_track_err_5] -> combine follower eta ksi/5(ksi_track_err_5)
  [eta_track_err_1] -> combine follower eta ksi/6(eta_track_err_1)
  [eta_track_err_2] -> combine follower eta ksi/7(eta_track_err_2)
  [eta_track_err_3] -> combine follower eta ksi/8(eta_track_err_3)
  [eta_track_err_4] -> combine follower eta ksi/9(eta_track_err_4)
  [eta_track_err_5] -> combine follower eta ksi/10(eta_track_err_5)
  combine follower eta ksi/1(ksi_track_err_vec) -> [ksi_track_err_vec]
  combine follower eta ksi/2(eta_track_err_vec) -> [eta_track_err_vec]
  Demux23/2 -> ksi_track_err_1/2
  Demux23/1 -> ksi_track_err_1/1
  Demux23/3 -> ksi_track_err_1/3
  Demux24/2 -> eta_track_err_1/2
  Demux24/1 -> eta_track_err_1/1
  Demux24/3 -> eta_track_err_1/3
  Demux25/2 -> ksi_track_err_2/2
  Demux25/1 -> ksi_track_err_2/1
  Demux25/3 -> ksi_track_err_2/3
  Demux26/1 -> eta_track_err_2/1
  Demux26/3 -> eta_track_err_2/3
  Demux26/2 -> eta_track_err_2/2
  Demux27/1 -> ksi_track_err_3/1
  Demux27/3 -> ksi_track_err_3/3
  Demux27/2 -> ksi_track_err_3/2
  Demux28/3 -> eta_track_err_3/3
  Demux28/2 -> eta_track_err_3/2
  Demux28/1 -> eta_track_err_3/1
  Demux29/3 -> ksi_track_err_4/3
  Demux29/2 -> ksi_track_err_4/2
  Demux29/1 -> ksi_track_err_4/1
  Demux30/3 -> eta_track_err_4/3
  Demux30/2 -> eta_track_err_4/2
  Demux30/1 -> eta_track_err_4/1
  Demux31/3 -> ksi_track_err_5/3
  Demux31/2 -> ksi_track_err_5/2
  Demux31/1 -> ksi_track_err_5/1
  Demux32/3 -> eta_track_err_5/3
  Demux32/2 -> eta_track_err_5/2
  Demux32/1 -> eta_track_err_5/1
  combine formation control input/1(eta_i_vec) -> Memory1/1
  Memory1/1 -> [eta_i_vec]
  combine formation control input/2(ksi_i_vec) -> Memory2/1
  Memory2/1 -> [ksi_i_vec]
  [ui] -> uav translational dynamics agent 1/2(ui)
  [Ri] -> uav translational dynamics agent 1/1(Ri)
  uav translational dynamics agent 1/1(dvi) -> follower etai Integrator agent 1/1
  uav translational dynamics agent 2/1(dvi) -> follower etai Integrator agent 2/1
  [ui] -> uav translational dynamics agent 2/2(ui)
  [Ri] -> uav translational dynamics agent 2/1(Ri)
  [ui] -> uav translational dynamics agent 3/2(ui)
  [Ri] -> uav translational dynamics agent 3/1(Ri)
  uav translational dynamics agent 3/1(dvi) -> follower etai Integrator agent 3/1
  [ui] -> uav translational dynamics agent 4/2(ui)
  [Ri] -> uav translational dynamics agent 4/1(Ri)
  uav translational dynamics agent 4/1(dvi) -> follower etai Integrator agent 4/1
  [ui] -> uav translational dynamics agent 5/2(ui)
  [Ri] -> uav translational dynamics agent 5/1(Ri)
  uav translational dynamics agent 5/1(dvi) -> follower etai Integrator agent 5/1
  [ui] -> cal Rci from ui/2(ui_vec)
  Constant191/1 -> cal Rci from ui/1(mi_vec)
  cal Rei/1(Rei) -> depart Re5/1(x), depart Re4/1(x), depart Re3/1(x), depart Re2/1(x), depart Re1/1(x), [Rei]
  depart Re2/1(y) -> Display65/1
  depart Re3/1(y) -> Display66/1
  depart Re1/1(y) -> Display64/1
  depart Re4/1(y) -> Display67/1
  Constant51/1 -> cal Rei/1(Qei)
  depart Re5/1(y) -> Display68/1
  [Rei] -> cal Ri/1(Rei)
  [Rci] -> cal Ri/2(Rci)
  cal Ri/1(Ri) -> [Ri]
  depart Rc5/1(y) -> Display25/1
  depart Rc2/1(y) -> Display22/1
  depart Rc3/1(y) -> Display23/1
  depart Rc4/1(y) -> Display24/1
  depart Rc1/1(y) -> Display6/1
  cal Rci from ui/1(Rci) -> [Rci], depart Rc5/1(x), depart Rc4/1(x), depart Rc3/1(x), depart Rc2/1(x), depart Rc1/1(x)
  [dp_vec] -> uav translational dynamics agent 1/3(dpi_vec)
  [dp_vec] -> uav translational dynamics agent 2/3(dpi_vec)
  [dp_vec] -> uav translational dynamics agent 3/3(dpi_vec)
  [dp_vec] -> uav translational dynamics agent 4/3(dpi_vec)
  [dp_vec] -> uav translational dynamics agent 5/3(dpi_vec)
  [Ri] -> cal virtual control sigma_v agent 1/2(Ri)
  [ui] -> cal virtual control sigma_v agent 1/3(ui)
  Constant92/1 -> cal virtual control sigma_v agent 1/1(c3v)
  [sigma_bar_v_vec] -> cal virtual control sigma_v agent 1/4(sigma_bar_v_vec)
  cal virtual control sigma_v agent 1/1(d_sigma_v_1) -> sigma_v Integrator 1/1
  sigma_v Integrator 1/1 -> [sigma_v_1]
  [sigma_bar_v_vec] -> cal virtual control sigma_v agent 2/4(sigma_bar_v_vec)
  sigma_v Integrator 2/1 -> [sigma_v_2]
  Constant93/1 -> cal virtual control sigma_v agent 2/1(c3v)
  [Ri] -> cal virtual control sigma_v agent 2/2(Ri)
  cal virtual control sigma_v agent 2/1(d_sigma_v_2) -> sigma_v Integrator 2/1
  [ui] -> cal virtual control sigma_v agent 2/3(ui)
  Constant94/1 -> cal virtual control sigma_v agent 3/1(c3v)
  cal virtual control sigma_v agent 3/1(d_sigma_v_3) -> sigma_v Integrator 3/1
  [ui] -> cal virtual control sigma_v agent 3/3(ui)
  [Ri] -> cal virtual control sigma_v agent 3/2(Ri)
  [sigma_bar_v_vec] -> cal virtual control sigma_v agent 3/4(sigma_bar_v_vec)
  sigma_v Integrator 3/1 -> [sigma_v_3]
  sigma_v Integrator 4/1 -> [sigma_v_4]
  [Ri] -> cal virtual control sigma_v agent 4/2(Ri)
  [sigma_bar_v_vec] -> cal virtual control sigma_v agent 4/4(sigma_bar_v_vec)
  [ui] -> cal virtual control sigma_v agent 4/3(ui)
  cal virtual control sigma_v agent 4/1(d_sigma_v_4) -> sigma_v Integrator 4/1
  Constant95/1 -> cal virtual control sigma_v agent 4/1(c3v)
  Constant96/1 -> cal virtual control sigma_v agent 5/1(c3v)
  [sigma_bar_v_vec] -> cal virtual control sigma_v agent 5/4(sigma_bar_v_vec)
  [Ri] -> cal virtual control sigma_v agent 5/2(Ri)
  [ui] -> cal virtual control sigma_v agent 5/3(ui)
  sigma_v Integrator 5/1 -> [sigma_v_5]
  cal virtual control sigma_v agent 5/1(d_sigma_v_5) -> sigma_v Integrator 5/1
  combine sigma_v/1(sigma_v_vec) -> [sigma_v_vec]
  [sigma_v_4] -> combine sigma_v/4(sigma_v_4)
  [sigma_v_3] -> combine sigma_v/3(sigma_v_3)
  [sigma_v_1] -> combine sigma_v/1(sigma_v_1)
  [sigma_v_5] -> combine sigma_v/5(sigma_v_5)
  [sigma_v_2] -> combine sigma_v/2(sigma_v_2)
  [eta_i_vec] -> cal combine sigma_bar_v/1(eta_i_vec)
  [sigma_v_vec] -> cal combine sigma_bar_v/2(sigma_v_vec)
  cal combine sigma_bar_v/1(sigma_bar_v_vec) -> [sigma_bar_v_vec]
  Demux12/3 -> d2_sigma_bar_v_est_1/3
  Demux12/2 -> d2_sigma_bar_v_est_1/2
  Demux8/3 -> d_sigma_bar_v_est_1/3
  Demux12/1 -> d2_sigma_bar_v_est_1/1
  Demux8/1 -> d_sigma_bar_v_est_1/1
  Demux8/2 -> d_sigma_bar_v_est_1/2
  cal differentiator d_sigma_bar_v_hat agent 1/1(Out1) -> Display35/1, [sigma_bar_v_est_1]
  cal differentiator d_sigma_bar_v_hat agent 1/2(Out2) -> Demux8/1, [d_sigma_bar_v_est_1], Display36/1
  cal differentiator d_sigma_bar_v_hat agent 1/3(Out3) -> Demux12/1, [d2_sigma_bar_v_est_1], Display37/1
  [sigma_bar_v_vec] -> cal differentiator d_sigma_bar_v_hat agent 1/1(x)
  cal differentiator d_sigma_bar_v_hat agent 2/1(Out1) -> Display38/1, [sigma_bar_v_est_2]
  [sigma_bar_v_vec] -> cal differentiator d_sigma_bar_v_hat agent 2/1(x)
  cal differentiator d_sigma_bar_v_hat agent 2/2(Out2) -> Demux3/1, [d_sigma_bar_v_est_2], Display39/1
  cal differentiator d_sigma_bar_v_hat agent 2/3(Out3) -> Demux2/1, [d2_sigma_bar_v_est_2], Display40/1
  Demux2/2 -> d2_sigma_bar_v_est_2/2
  Demux2/3 -> d2_sigma_bar_v_est_2/3
  Demux3/2 -> d_sigma_bar_v_est_2/2
  Demux2/1 -> d2_sigma_bar_v_est_2/1
  Demux3/1 -> d_sigma_bar_v_est_2/1
  Demux3/3 -> d_sigma_bar_v_est_2/3
  Demux5/1 -> d_sigma_bar_v_est_3/1
  Demux5/3 -> d_sigma_bar_v_est_3/3
  Demux4/2 -> d2_sigma_bar_v_est_3/2
  Demux4/3 -> d2_sigma_bar_v_est_3/3
  Demux5/2 -> d_sigma_bar_v_est_3/2
  Demux4/1 -> d2_sigma_bar_v_est_3/1
  cal differentiator d_sigma_bar_v_hat agent 3/3(Out3) -> Demux4/1, [d2_sigma_bar_v_est_3], Display43/1
  cal differentiator d_sigma_bar_v_hat agent 3/2(Out2) -> Demux5/1, [d_sigma_bar_v_est_3], Display42/1
  cal differentiator d_sigma_bar_v_hat agent 3/1(Out1) -> Display41/1, [sigma_bar_v_est_3]
  [sigma_bar_v_vec] -> cal differentiator d_sigma_bar_v_hat agent 3/1(x)
  cal differentiator d_sigma_bar_v_hat agent 4/3(Out3) -> Demux6/1, [d2_sigma_bar_v_est_4], Display46/1
  Demux6/1 -> d2_sigma_bar_v_est_4/1
  Demux6/3 -> d2_sigma_bar_v_est_4/3
  Demux7/2 -> d_sigma_bar_v_est_4/2
  Demux6/2 -> d2_sigma_bar_v_est_4/2
  Demux7/3 -> d_sigma_bar_v_est_4/3
  Demux7/1 -> d_sigma_bar_v_est_4/1
  cal differentiator d_sigma_bar_v_hat agent 4/1(Out1) -> Display44/1, [sigma_bar_v_est_4]
  cal differentiator d_sigma_bar_v_hat agent 4/2(Out2) -> Demux7/1, [d_sigma_bar_v_est_4], Display45/1
  [sigma_bar_v_vec] -> cal differentiator d_sigma_bar_v_hat agent 4/1(x)
  cal differentiator d_sigma_bar_v_hat agent 5/1(Out1) -> Display47/1, [sigma_bar_v_est_5]
  cal differentiator d_sigma_bar_v_hat agent 5/2(Out2) -> Demux10/1, [d_sigma_bar_v_est_5], Display48/1
  [sigma_bar_v_vec] -> cal differentiator d_sigma_bar_v_hat agent 5/1(x)
  Demux10/3 -> d_sigma_bar_v_est_5/3
  Demux9/2 -> d2_sigma_bar_v_est_5/2
  Demux10/2 -> d_sigma_bar_v_est_5/2
  Demux9/1 -> d2_sigma_bar_v_est_5/1
  cal differentiator d_sigma_bar_v_hat agent 5/3(Out3) -> Demux9/1, [d2_sigma_bar_v_est_5], Display49/1
  Demux10/1 -> d_sigma_bar_v_est_5/1
  Demux9/3 -> d2_sigma_bar_v_est_5/3
  [d_sigma_bar_v_est_5] -> combine d_sigma_bar_v_est/5(d_sigma_bar_v_est_5)
  [d_sigma_bar_v_est_2] -> combine d_sigma_bar_v_est/2(d_sigma_bar_v_est_2)
  [d_sigma_bar_v_est_1] -> combine d_sigma_bar_v_est/1(d_sigma_bar_v_est_1)
  [d_sigma_bar_v_est_4] -> combine d_sigma_bar_v_est/4(d_sigma_bar_v_est_4)
  [d_sigma_bar_v_est_3] -> combine d_sigma_bar_v_est/3(d_sigma_bar_v_est_3)
  combine d_sigma_bar_v_est/1(d_sigma_bar_v_vec) -> [d_sigma_bar_v_vec]
  trans to column21/1(y) -> [sigma_bar_v_tilt_squ_1_1], Display51/1
  Constant100/1 -> Mux20/2
  Constant97/1 -> Mux20/3
  Interpreted MATLAB Function21/1 -> trans to column21/1(x)
  [sigma_bar_v_tilt_vec] -> choose ksi_est_err 21/1(x)
  choose ksi_est_err 21/1(y) -> cal abs 21/1(x)
  Constant98/1 -> Mux19/2
  cal abs 22/1(y) -> Mux19/1
  choose ksi_est_err 22/1(y) -> cal abs 22/1(x)
  Interpreted MATLAB Function20/1 -> trans to column20/1(x)
  cal abs 21/1(y) -> Mux20/1
  Mux19/1 -> Interpreted MATLAB Function20/1
  trans to column20/1(y) -> [sigma_bar_v_tilt_squ_2_1], Display50/1
  Constant99/1 -> Mux19/3
  Mux20/1 -> Interpreted MATLAB Function21/1
  [sigma_bar_v_tilt_vec] -> choose ksi_est_err 22/1(x)
  cal theta_sigma_bar_v_tilt agent 1/1(theta_sigma_bar_v_tilt_1_1) -> [theta_sigma_bar_v_tilt_1_1]
  [sigma_bar_v_tilt_squ_1_1] -> cal theta_sigma_bar_v_tilt agent 1/2(sigma_bar_v_tilt_squ_1_1)
  cal theta_sigma_bar_v_tilt agent 1/2(theta_sigma_bar_v_tilt_2_1) -> [theta_sigma_bar_v_tilt_2_1]
  [sigma_bar_v_tilt_vec] -> cal theta_sigma_bar_v_tilt agent 1/4(sigma_bar_v_tilt_vec)
  [sigma_bar_v_tilt_squ_2_1] -> cal theta_sigma_bar_v_tilt agent 1/3(sigma_bar_v_tilt_squ_2_1)
  Constant101/1 -> cal theta_sigma_bar_v_tilt agent 1/1(alfa_theta)
  Constant103/1 -> cal theta_sigma_bar_v_tilt agent 2/1(alfa_theta)
  [sigma_bar_v_tilt_vec] -> cal theta_sigma_bar_v_tilt agent 2/4(sigma_bar_v_tilt_vec)
  [sigma_bar_v_tilt_squ_1_2] -> cal theta_sigma_bar_v_tilt agent 2/2(sigma_bar_v_tilt_squ_1_2)
  trans to column23/1(y) -> [sigma_bar_v_tilt_squ_1_2], Display53/1
  Interpreted MATLAB Function23/1 -> trans to column23/1(x)
  Mux22/1 -> Interpreted MATLAB Function23/1
  Constant106/1 -> Mux21/3
  cal theta_sigma_bar_v_tilt agent 2/1(theta_sigma_bar_v_tilt_1_2) -> [theta_sigma_bar_v_tilt_1_2]
  Constant102/1 -> Mux22/2
  trans to column22/1(y) -> [sigma_bar_v_tilt_squ_2_2], Display52/1
  Interpreted MATLAB Function22/1 -> trans to column22/1(x)
  cal abs 23/1(y) -> Mux22/1
  Constant104/1 -> Mux22/3
  Mux21/1 -> Interpreted MATLAB Function22/1
  choose ksi_est_err 24/1(y) -> cal abs 24/1(x)
  cal abs 24/1(y) -> Mux21/1
  choose ksi_est_err 23/1(y) -> cal abs 23/1(x)
  [sigma_bar_v_tilt_vec] -> choose ksi_est_err 24/1(x)
  [sigma_bar_v_tilt_squ_2_2] -> cal theta_sigma_bar_v_tilt agent 2/3(sigma_bar_v_tilt_squ_2_2)
  Constant105/1 -> Mux21/2
  [sigma_bar_v_tilt_vec] -> choose ksi_est_err 23/1(x)
  cal theta_sigma_bar_v_tilt agent 2/2(theta_sigma_bar_v_tilt_2_2) -> [theta_sigma_bar_v_tilt_2_2]
  [sigma_bar_v_tilt_vec] -> choose ksi_est_err 25/1(x)
  cal theta_sigma_bar_v_tilt agent 3/2(theta_sigma_bar_v_tilt_2_3) -> [theta_sigma_bar_v_tilt_2_3]
  Constant110/1 -> Mux23/2
  [sigma_bar_v_tilt_squ_2_3] -> cal theta_sigma_bar_v_tilt agent 3/3(sigma_bar_v_tilt_squ_2_3)
  [sigma_bar_v_tilt_vec] -> choose ksi_est_err 26/1(x)
  choose ksi_est_err 25/1(y) -> cal abs 25/1(x)
  Mux23/1 -> Interpreted MATLAB Function24/1
  choose ksi_est_err 26/1(y) -> cal abs 26/1(x)
  Constant109/1 -> Mux24/3
  cal abs 25/1(y) -> Mux24/1
  Interpreted MATLAB Function24/1 -> trans to column24/1(x)
  Constant107/1 -> Mux24/2
  Mux24/1 -> Interpreted MATLAB Function25/1
  cal theta_sigma_bar_v_tilt agent 3/1(theta_sigma_bar_v_tilt_1_3) -> [theta_sigma_bar_v_tilt_1_3]
  Constant111/1 -> Mux23/3
  Constant108/1 -> cal theta_sigma_bar_v_tilt agent 3/1(alfa_theta)
  trans to column24/1(y) -> [sigma_bar_v_tilt_squ_2_3], Display54/1
  [sigma_bar_v_tilt_squ_1_3] -> cal theta_sigma_bar_v_tilt agent 3/2(sigma_bar_v_tilt_squ_1_3)
  trans to column25/1(y) -> [sigma_bar_v_tilt_squ_1_3], Display55/1
  Interpreted MATLAB Function25/1 -> trans to column25/1(x)
  [sigma_bar_v_tilt_vec] -> cal theta_sigma_bar_v_tilt agent 3/4(sigma_bar_v_tilt_vec)
  cal abs 26/1(y) -> Mux23/1
  cal abs 28/1(y) -> Mux25/1
  trans to column27/1(y) -> [sigma_bar_v_tilt_squ_1_4], Display57/1
  Interpreted MATLAB Function27/1 -> trans to column27/1(x)
  Constant113/1 -> cal theta_sigma_bar_v_tilt agent 4/1(alfa_theta)
  [sigma_bar_v_tilt_squ_1_4] -> cal theta_sigma_bar_v_tilt agent 4/2(sigma_bar_v_tilt_squ_1_4)
  Constant116/1 -> Mux25/3
  trans to column26/1(y) -> [sigma_bar_v_tilt_squ_2_4], Display56/1
  Constant112/1 -> Mux26/2
  Mux26/1 -> Interpreted MATLAB Function27/1
  [sigma_bar_v_tilt_vec] -> cal theta_sigma_bar_v_tilt agent 4/4(sigma_bar_v_tilt_vec)
  Constant114/1 -> Mux26/3
  cal abs 27/1(y) -> Mux26/1
  cal theta_sigma_bar_v_tilt agent 4/1(theta_sigma_bar_v_tilt_1_4) -> [theta_sigma_bar_v_tilt_1_4]
  Constant115/1 -> Mux25/2
  choose ksi_est_err 27/1(y) -> cal abs 27/1(x)
  choose ksi_est_err 28/1(y) -> cal abs 28/1(x)
  Interpreted MATLAB Function26/1 -> trans to column26/1(x)
  cal theta_sigma_bar_v_tilt agent 4/2(theta_sigma_bar_v_tilt_2_4) -> [theta_sigma_bar_v_tilt_2_4]
  [sigma_bar_v_tilt_vec] -> choose ksi_est_err 28/1(x)
  [sigma_bar_v_tilt_squ_2_4] -> cal theta_sigma_bar_v_tilt agent 4/3(sigma_bar_v_tilt_squ_2_4)
  [sigma_bar_v_tilt_vec] -> choose ksi_est_err 27/1(x)
  Mux25/1 -> Interpreted MATLAB Function26/1
  [sigma_bar_v_tilt_squ_2_5] -> cal theta_sigma_bar_v_tilt agent 5/3(sigma_bar_v_tilt_squ_2_5)
  choose ksi_est_err 29/1(y) -> cal abs 29/1(x)
  Interpreted MATLAB Function28/1 -> trans to column28/1(x)
  choose ksi_est_err 30/1(y) -> cal abs 30/1(x)
  Constant120/1 -> Mux27/2
  cal theta_sigma_bar_v_tilt agent 5/2(theta_sigma_bar_v_tilt_2_5) -> [theta_sigma_bar_v_tilt_2_5]
  [sigma_bar_v_tilt_vec] -> choose ksi_est_err 29/1(x)
  cal theta_sigma_bar_v_tilt agent 5/1(theta_sigma_bar_v_tilt_1_5) -> [theta_sigma_bar_v_tilt_1_5]
  [sigma_bar_v_tilt_vec] -> choose ksi_est_err 30/1(x)
  Constant119/1 -> Mux28/3
  trans to column28/1(y) -> [sigma_bar_v_tilt_squ_2_5], Display58/1
  Mux28/1 -> Interpreted MATLAB Function29/1
  Constant117/1 -> Mux28/2
  cal abs 29/1(y) -> Mux28/1
  [sigma_bar_v_tilt_squ_1_5] -> cal theta_sigma_bar_v_tilt agent 5/2(sigma_bar_v_tilt_squ_1_5)
  Mux27/1 -> Interpreted MATLAB Function28/1
  Constant121/1 -> Mux27/3
  Interpreted MATLAB Function29/1 -> trans to column29/1(x)
  [sigma_bar_v_tilt_vec] -> cal theta_sigma_bar_v_tilt agent 5/4(sigma_bar_v_tilt_vec)
  Constant118/1 -> cal theta_sigma_bar_v_tilt agent 5/1(alfa_theta)
  trans to column29/1(y) -> [sigma_bar_v_tilt_squ_1_5], Display59/1
  cal abs 30/1(y) -> Mux27/1
  combine theta_sigma_bar_v_tilt/1(theta_sigma_bar_v_tilt_1_vec) -> [theta_sigma_bar_v_tilt_1_vec]
  [theta_sigma_bar_v_tilt_2_1] -> combine theta_sigma_bar_v_tilt/6(theta_sigma_bar_v_tilt_2_1)
  [theta_sigma_bar_v_tilt_1_4] -> combine theta_sigma_bar_v_tilt/4(theta_sigma_bar_v_tilt_1_4)
  [theta_sigma_bar_v_tilt_2_2] -> combine theta_sigma_bar_v_tilt/7(theta_sigma_bar_v_tilt_2_2)
  [theta_sigma_bar_v_tilt_1_2] -> combine theta_sigma_bar_v_tilt/2(theta_sigma_bar_v_tilt_1_2)
  [theta_sigma_bar_v_tilt_2_5] -> combine theta_sigma_bar_v_tilt/10(theta_sigma_bar_v_tilt_2_5)
  [theta_sigma_bar_v_tilt_2_4] -> combine theta_sigma_bar_v_tilt/9(theta_sigma_bar_v_tilt_2_4)
  combine theta_sigma_bar_v_tilt/2(theta_sigma_bar_v_tilt_2_vec) -> [theta_sigma_bar_v_tilt_2_vec]
  [theta_sigma_bar_v_tilt_1_1] -> combine theta_sigma_bar_v_tilt/1(theta_sigma_bar_v_tilt_1_1)
  [theta_sigma_bar_v_tilt_2_3] -> combine theta_sigma_bar_v_tilt/8(theta_sigma_bar_v_tilt_2_3)
  [theta_sigma_bar_v_tilt_1_5] -> combine theta_sigma_bar_v_tilt/5(theta_sigma_bar_v_tilt_1_5)
  [theta_sigma_bar_v_tilt_1_3] -> combine theta_sigma_bar_v_tilt/3(theta_sigma_bar_v_tilt_1_3)
  Constant122/1 -> cal sigma_bar_v_hat agent 1/1(c1v)
  Constant123/1 -> cal sigma_bar_v_hat agent 1/2(c2v)
  [theta_sigma_bar_v_tilt_1_vec] -> cal sigma_bar_v_hat agent 1/3(theta_sigma_bar_v_tilt_1_vec)
  [theta_sigma_bar_v_tilt_2_vec] -> cal sigma_bar_v_hat agent 1/4(theta_sigma_bar_v_tilt_2_vec)
  [d_sigma_bar_v_vec] -> cal sigma_bar_v_hat agent 1/5(d_sigma_bar_v_vec)
  cal sigma_bar_v_hat agent 1/1(d_sigma_bar_v_hat_1) -> sigma_bar_v_hat Integrator 1/1
  [theta_sigma_bar_v_tilt_2_vec] -> cal sigma_bar_v_hat agent 2/4(theta_sigma_bar_v_tilt_2_vec)
  Constant125/1 -> cal sigma_bar_v_hat agent 2/2(c2v)
  cal sigma_bar_v_hat agent 2/1(d_sigma_bar_v_hat_2) -> sigma_bar_v_hat Integrator 2/1
  [d_sigma_bar_v_vec] -> cal sigma_bar_v_hat agent 2/5(d_sigma_bar_v_vec)
  [theta_sigma_bar_v_tilt_1_vec] -> cal sigma_bar_v_hat agent 2/3(theta_sigma_bar_v_tilt_1_vec)
  Constant124/1 -> cal sigma_bar_v_hat agent 2/1(c1v)
  Constant126/1 -> cal sigma_bar_v_hat agent 3/1(c1v)
  [theta_sigma_bar_v_tilt_2_vec] -> cal sigma_bar_v_hat agent 3/4(theta_sigma_bar_v_tilt_2_vec)
  cal sigma_bar_v_hat agent 3/1(d_sigma_bar_v_hat_3) -> sigma_bar_v_hat Integrator 3/1
  [d_sigma_bar_v_vec] -> cal sigma_bar_v_hat agent 3/5(d_sigma_bar_v_vec)
  Constant127/1 -> cal sigma_bar_v_hat agent 3/2(c2v)
  [theta_sigma_bar_v_tilt_1_vec] -> cal sigma_bar_v_hat agent 3/3(theta_sigma_bar_v_tilt_1_vec)
  [d_sigma_bar_v_vec] -> cal sigma_bar_v_hat agent 4/5(d_sigma_bar_v_vec)
  [theta_sigma_bar_v_tilt_1_vec] -> cal sigma_bar_v_hat agent 4/3(theta_sigma_bar_v_tilt_1_vec)
  Constant139/1 -> cal sigma_bar_v_hat agent 4/2(c2v)
  cal sigma_bar_v_hat agent 4/1(d_sigma_bar_v_hat_4) -> sigma_bar_v_hat Integrator 4/1
  [theta_sigma_bar_v_tilt_2_vec] -> cal sigma_bar_v_hat agent 4/4(theta_sigma_bar_v_tilt_2_vec)
  Constant128/1 -> cal sigma_bar_v_hat agent 4/1(c1v)
  [sigma_bar_v_hat_5] -> combine sigma_bar_v_hat/5(sigma_bar_v_hat_5)
  [sigma_bar_v_hat_4] -> combine sigma_bar_v_hat/4(sigma_bar_v_hat_4)
  [sigma_bar_v_hat_3] -> combine sigma_bar_v_hat/3(sigma_bar_v_hat_3)
  combine sigma_bar_v_hat/1(sigma_bar_v_hat_vec) -> [sigma_bar_v_hat_vec]
  cal combine sigma_bar_v_tilt/1(sigma_bar_v_tilt_vec) -> [sigma_bar_v_tilt_vec]
  [sigma_bar_v_vec] -> cal combine sigma_bar_v_tilt/1(sigma_bar_v_vec)
  [sigma_bar_v_hat_vec] -> cal combine sigma_bar_v_tilt/2(sigma_bar_v_hat_vec)
  [sigma_bar_v_hat_2] -> combine sigma_bar_v_hat/2(sigma_bar_v_hat_2)
  [sigma_bar_v_hat_1] -> combine sigma_bar_v_hat/1(sigma_bar_v_hat_1)
  sigma_bar_v_hat Integrator 1/1 -> [sigma_bar_v_hat_1]
  sigma_bar_v_hat Integrator 2/1 -> [sigma_bar_v_hat_2]
  sigma_bar_v_hat Integrator 3/1 -> [sigma_bar_v_hat_3]
  sigma_bar_v_hat Integrator 4/1 -> [sigma_bar_v_hat_4]
  sigma_bar_v_hat Integrator 5/1 -> [sigma_bar_v_hat_5]
  [d_sigma_bar_v_vec] -> cal sigma_bar_v_hat agent 5/5(d_sigma_bar_v_vec)
  [theta_sigma_bar_v_tilt_2_vec] -> cal sigma_bar_v_hat agent 5/4(theta_sigma_bar_v_tilt_2_vec)
  cal sigma_bar_v_hat agent 5/1(d_sigma_bar_v_hat_5) -> sigma_bar_v_hat Integrator 5/1
  [theta_sigma_bar_v_tilt_1_vec] -> cal sigma_bar_v_hat agent 5/3(theta_sigma_bar_v_tilt_1_vec)
  Constant141/1 -> cal sigma_bar_v_hat agent 5/2(c2v)
  Constant140/1 -> cal sigma_bar_v_hat agent 5/1(c1v)
  Constant142/1 -> cal dp_hat agent 1/1(c3v)
  [d_sigma_bar_v_vec] -> cal dp_hat agent 1/2(d_sigma_bar_v_vec)
  [sigma_bar_v_hat_vec] -> cal dp_hat agent 1/3(sigma_bar_v_hat_vec)
  cal dp_hat agent 1/1(dp_hat_1) -> [dp_hat_1]
  cal dp_hat agent 2/1(dp_hat_2) -> [dp_hat_2]
  [d_sigma_bar_v_vec] -> cal dp_hat agent 2/2(d_sigma_bar_v_vec)
  Constant143/1 -> cal dp_hat agent 2/1(c3v)
  [sigma_bar_v_hat_vec] -> cal dp_hat agent 2/3(sigma_bar_v_hat_vec)
  [sigma_bar_v_hat_vec] -> cal dp_hat agent 3/3(sigma_bar_v_hat_vec)
  Constant144/1 -> cal dp_hat agent 3/1(c3v)
  [d_sigma_bar_v_vec] -> cal dp_hat agent 3/2(d_sigma_bar_v_vec)
  cal dp_hat agent 3/1(dp_hat_3) -> [dp_hat_3]
  cal dp_hat agent 4/1(dp_hat_4) -> [dp_hat_4]
  [d_sigma_bar_v_vec] -> cal dp_hat agent 4/2(d_sigma_bar_v_vec)
  Constant145/1 -> cal dp_hat agent 4/1(c3v)
  [sigma_bar_v_hat_vec] -> cal dp_hat agent 4/3(sigma_bar_v_hat_vec)
  cal dp_hat agent 5/1(dp_hat_5) -> [dp_hat_5]
  [sigma_bar_v_hat_vec] -> cal dp_hat agent 5/3(sigma_bar_v_hat_vec)
  Constant146/1 -> cal dp_hat agent 5/1(c3v)
  [d_sigma_bar_v_vec] -> cal dp_hat agent 5/2(d_sigma_bar_v_vec)
  combine dp_hat/1(dp_hat_vec) -> [dp_hat_vec]
  [dp_hat_1] -> combine dp_hat/1(dp_hat_1)
  [dp_hat_4] -> combine dp_hat/4(dp_hat_4)
  [dp_hat_3] -> combine dp_hat/3(dp_hat_3)
  [dp_hat_5] -> combine dp_hat/5(dp_hat_5)
  [dp_hat_2] -> combine dp_hat/2(dp_hat_2)
  cal ui agent 1/1(ui_1) -> [ui_1]
  [ui_5] -> combine ui/5(ui_5)
  [ui_2] -> combine ui/2(ui_2)
  [ui_1] -> combine ui/1(ui_1)
  [ui_4] -> combine ui/4(ui_4)
  [ui_3] -> combine ui/3(ui_3)
  [dp_vec] -> cal disturbance observation error dp_tilt/1(dp_vec)
  [dp_hat_vec] -> cal disturbance observation error dp_tilt/2(dp_hat_vec)
  cal disturbance observation error dp_tilt/1(dp_tilt_vec) -> [dp_tilt_vec]
  combine ui/1(ui) -> [ui]
  Phi_sec_sigma_i agent 1/1(Phi_sec_sigma_1) -> [Phi_sec_sigma_1]
  Phi_sec_sigma_i agent 5/1(Phi_sec_sigma_5) -> [Phi_sec_sigma_5]
  combine Phi_sec_sigma_i/1(Phi_sec_sigma_vec) -> Memory/1
  [Phi_sec_sigma_5] -> combine Phi_sec_sigma_i/5(Phi_sec_sigma_5)
  [Phi_sec_sigma_1] -> combine Phi_sec_sigma_i/1(Phi_sec_sigma_1)
  [sigmai_vec] -> Phi_sec_sigma_i agent 2/1(sigma_i_vec)
  [Phi_sec_sigma_4] -> combine Phi_sec_sigma_i/4(Phi_sec_sigma_4)
  Phi_sec_sigma_i agent 4/1(Phi_sec_sigma_4) -> [Phi_sec_sigma_4]
  Phi_sec_sigma_i agent 3/1(Phi_sec_sigma_3) -> [Phi_sec_sigma_3]
  [sigmai_vec] -> Phi_sec_sigma_i agent 5/1(sigma_i_vec)
  Phi_sec_sigma_i agent 2/1(Phi_sec_sigma_2) -> [Phi_sec_sigma_2]
  [sigmai_vec] -> Phi_sec_sigma_i agent 1/1(sigma_i_vec)
  [Phi_sec_sigma_2] -> combine Phi_sec_sigma_i/2(Phi_sec_sigma_2)
  [Phi_sec_sigma_3] -> combine Phi_sec_sigma_i/3(Phi_sec_sigma_3)
  [sigmai_vec] -> Phi_sec_sigma_i agent 3/1(sigma_i_vec)
  Memory/1 -> [Phi_sec_sigma_vec]
  [sigmai_vec] -> Phi_sec_sigma_i agent 4/1(sigma_i_vec)
  Constant2/1 -> update betai agent 1/3(Mii)
  [u0] -> update betai agent 3/5(u0)
  [tsim] -> update betai agent 4/4(tsim)
  [rho_hat_vec] -> update betai agent 2/6(rho_hat_vec)
  Constant4/1 -> update betai agent 2/2(Wij)
  Constant13/1 -> update betai agent 5/3(Mii)
  Constant3/1 -> update betai agent 2/1(eps0)
  [u0] -> update betai agent 2/5(u0)
  beta_hat Integrator 1/1 -> [beta_hat_1]
  beta_hat Integrator 2/1 -> [beta_hat_2]
  Constant12/1 -> update betai agent 5/2(Wij)
  [u0] -> update betai agent 5/5(u0)
  [rho_hat_vec] -> update betai agent 1/6(rho_hat_vec)
  Constant14/1 -> update betai agent 5/1(eps0)
  [tsim] -> update betai agent 2/4(tsim)
  combine beta_hat/1(beta_hat_vec) -> Memory4/1
  [beta_hat_5] -> combine beta_hat/5(beta_hat_5)
  [beta_hat_3] -> combine beta_hat/3(beta_hat_3)
  [beta_hat_4] -> combine beta_hat/4(beta_hat_4)
  [beta_hat_2] -> combine beta_hat/2(beta_hat_2)
  Memory4/1 -> [beta_hat_vec]
  beta_hat Integrator 5/1 -> [beta_hat_5]
  beta_hat Integrator 4/1 -> [beta_hat_4]
  update betai agent 5/1(d_beta_hat_5) -> beta_hat Integrator 5/1
  [beta_hat_1] -> combine beta_hat/1(beta_hat_1)
  Constant9/1 -> update betai agent 4/1(eps0)
  Constant10/1 -> update betai agent 4/2(Wij)
  [tsim] -> update betai agent 3/4(tsim)
  Constant11/1 -> update betai agent 4/3(Mii)
  [rho_hat_vec] -> update betai agent 4/6(rho_hat_vec)
  Constant8/1 -> update betai agent 3/3(Mii)
  beta_hat Integrator 3/1 -> [beta_hat_3]
  Constant7/1 -> update betai agent 3/2(Wij)
  Constant1/1 -> update betai agent 1/2(Wij)
  [tsim] -> update betai agent 1/4(tsim)
  update betai agent 2/1(d_beta_hat_2) -> beta_hat Integrator 2/1
  [u0] -> update betai agent 1/5(u0)
  [tsim] -> update betai agent 5/4(tsim)
  update betai agent 3/1(d_beta_hat_3) -> beta_hat Integrator 3/1
  update betai agent 1/1(d_beta_hat_1) -> beta_hat Integrator 1/1
  [u0] -> update betai agent 4/5(u0)
  Constant/1 -> update betai agent 1/1(eps0)
  Constant6/1 -> update betai agent 3/1(eps0)
  [rho_hat_vec] -> update betai agent 3/6(rho_hat_vec)
  Constant5/1 -> update betai agent 2/3(Mii)
  [rho_hat_vec] -> update betai agent 5/6(rho_hat_vec)
  update betai agent 4/1(d_beta_hat_4) -> beta_hat Integrator 4/1
  update sigmai agent 3/1(d_sigmai_3) -> sigmai Integrator 3/1
  [beta_hat_vec] -> update sigmai agent 3/8(beta_hat_vec)
  [sigmai_4] -> combine betai1/4(sigmai_4)
  Constant19/1 -> update sigmai agent 1/5(Mii)
  Constant33/1 -> update sigmai agent 4/4(Wij)
  [Phi_sec_sigma_vec] -> update sigmai agent 1/10(Phi_sec_sigma_vec)
  Constant31/1 -> update sigmai agent 4/2(lam0)
  Memory5/1 -> [sigmai_vec]
  [Phi_sec_sigma_vec] -> update sigmai agent 5/10(Phi_sec_sigma_vec)
  Constant39/1 -> update sigmai agent 5/5(Mii)
  sigmai Integrator 5/1 -> [sigmai_5]
  Constant37/1 -> update sigmai agent 5/3(eps0)
  Constant38/1 -> update sigmai agent 5/4(Wij)
  update sigmai agent 5/1(d_sigmai_5) -> sigmai Integrator 5/1
  Constant26/1 -> update sigmai agent 3/2(lam0)
  [beta_hat_vec] -> update sigmai agent 5/8(beta_hat_vec)
  [u0] -> update sigmai agent 5/7(u0)
  [u0] -> update sigmai agent 4/7(u0)
  Constant32/1 -> update sigmai agent 4/3(eps0)
  sigmai Integrator 4/1 -> [sigmai_4]
  combine betai1/1(sigmai_vec) -> Memory5/1
  [tsim] -> update sigmai agent 4/6(tsim)
  [Phi_sec_sigma_vec] -> update sigmai agent 3/10(Phi_sec_sigma_vec)
  Constant28/1 -> update sigmai agent 3/4(Wij)
  [tsim] -> update sigmai agent 3/6(tsim)
  [rho_hat_vec] -> update sigmai agent 4/9(rho_hat_vec)
  [u0] -> update sigmai agent 2/7(u0)
  Constant34/1 -> update sigmai agent 4/5(Mii)
  [sigmai_3] -> combine betai1/3(sigmai_3)
  Constant22/1 -> update sigmai agent 2/3(eps0)
  [Phi_sec_sigma_vec] -> update sigmai agent 2/10(Phi_sec_sigma_vec)
  sigmai Integrator 1/1 -> [sigmai_1]
  update sigmai agent 2/1(d_sigmai_2) -> sigmai Integrator 2/1
  [tsim] -> update sigmai agent 2/6(tsim)
  [sigmai_5] -> combine betai1/5(sigmai_5)
  sigmai Integrator 3/1 -> [sigmai_3]
  [rho_hat_vec] -> update sigmai agent 2/9(rho_hat_vec)
  Constant24/1 -> update sigmai agent 2/5(Mii)
  Constant27/1 -> update sigmai agent 3/3(eps0)
  [beta_hat_vec] -> update sigmai agent 2/8(beta_hat_vec)
  Constant23/1 -> update sigmai agent 2/4(Wij)
  [u0] -> update sigmai agent 1/7(u0)
  Constant18/1 -> update sigmai agent 1/4(Wij)
  Constant17/1 -> update sigmai agent 1/3(eps0)
  [sigmai_2] -> combine betai1/2(sigmai_2)
  [tsim] -> update sigmai agent 1/6(tsim)
  [rho_hat_vec] -> update sigmai agent 3/9(rho_hat_vec)
  [rho_hat_vec] -> update sigmai agent 1/9(rho_hat_vec)
  Constant21/1 -> update sigmai agent 2/2(lam0)
  Constant15/1 -> update sigmai agent 1/1(kai0)
  Constant16/1 -> update sigmai agent 1/2(lam0)
  Constant35/1 -> update sigmai agent 5/1(kai0)
  Constant36/1 -> update sigmai agent 5/2(lam0)
  [beta_hat_vec] -> update sigmai agent 1/8(beta_hat_vec)
  [tsim] -> update sigmai agent 5/6(tsim)
  [beta_hat_vec] -> update sigmai agent 4/8(beta_hat_vec)
  sigmai Integrator 2/1 -> [sigmai_2]
  Constant20/1 -> update sigmai agent 2/1(kai0)
  [u0] -> update sigmai agent 3/7(u0)
  Constant29/1 -> update sigmai agent 3/5(Mii)
  Constant30/1 -> update sigmai agent 4/1(kai0)
  [Phi_sec_sigma_vec] -> update sigmai agent 4/10(Phi_sec_sigma_vec)
  [sigmai_1] -> combine betai1/1(sigmai_1)
  Constant25/1 -> update sigmai agent 3/1(kai0)
  update sigmai agent 1/1(d_sigmai_1) -> sigmai Integrator 1/1
  update sigmai agent 4/1(d_sigmai_4) -> sigmai Integrator 4/1
  [rho_hat_vec] -> update sigmai agent 5/9(rho_hat_vec)
  rho_hat agent 5/1(rho_hat_5) -> [rho_hat_5]
  [rho_hat_2] -> combine rho_hat/2(rho_hat_2)
  [rho_hat_vec] -> cal rho_err_vec/2(rho_hat_vec)
  Constant40/1 -> rho_hat agent 1/1(lam0)
  Memory6/1 -> [rho_hat_vec]
  Constant41/1 -> rho_hat agent 2/1(lam0)
  [rho_hat_5] -> combine rho_hat/5(rho_hat_5)
  rho_hat agent 2/1(rho_hat_2) -> [rho_hat_2]
  [rho_hat_1] -> combine rho_hat/1(rho_hat_1)
  rho_hat agent 3/1(rho_hat_3) -> [rho_hat_3]
  Constant44/1 -> rho_hat agent 5/1(lam0)
  [sigmai_vec] -> rho_hat agent 4/2(sigmai_vec)
  Constant43/1 -> rho_hat agent 4/1(lam0)
  [sigmai_vec] -> rho_hat agent 1/2(sigmai_vec)
  combine rho_hat/1(rho_hat_vec) -> Memory6/1
  Constant42/1 -> rho_hat agent 3/1(lam0)
  rho_hat agent 4/1(rho_hat_4) -> [rho_hat_4]
  [rho_hat_4] -> combine rho_hat/4(rho_hat_4)
  [sigmai_vec] -> rho_hat agent 5/2(sigmai_vec)
  [rho_hat_3] -> combine rho_hat/3(rho_hat_3)
  cal rho_err_vec/1(rho_err_vec) -> [rho_err_vec]
  [u0] -> cal rho_err_vec/1(u0)
  [sigmai_vec] -> rho_hat agent 3/2(sigmai_vec)
  rho_hat agent 1/1(rho_hat_1) -> [rho_hat_1]
  [sigmai_vec] -> rho_hat agent 2/2(sigmai_vec)
  cal ui agent 2/1(ui_2) -> [ui_2]
  cal ui agent 3/1(ui_3) -> [ui_3]
  cal ui agent 4/1(ui_4) -> [ui_4]
  cal ui agent 5/1(ui_5) -> [ui_5]
  Memory7/1 -> [ksi_ld_hat_vec]
  [ksi_i_vec] -> cal err_pos_i agent 1/2(ksi_i_vec)
  [ksi_ld_hat_vec] -> cal err_pos_i agent 1/3(ksi_ld_hat_vec)
  cal err_pos_i agent 1/1(err_pos_1) -> [err_pos_1]
  cal err_pos_i agent 2/1(err_pos_2) -> [err_pos_2]
  [ksi_i_vec] -> cal err_pos_i agent 2/2(ksi_i_vec)
  [ksi_ld_hat_vec] -> cal err_pos_i agent 2/3(ksi_ld_hat_vec)
  [ksi_ld_hat_vec] -> cal err_pos_i agent 3/3(ksi_ld_hat_vec)
  [ksi_i_vec] -> cal err_pos_i agent 3/2(ksi_i_vec)
  cal err_pos_i agent 3/1(err_pos_3) -> [err_pos_3]
  [ksi_i_vec] -> cal err_pos_i agent 4/2(ksi_i_vec)
  [ksi_ld_hat_vec] -> cal err_pos_i agent 4/3(ksi_ld_hat_vec)
  cal err_pos_i agent 4/1(err_pos_4) -> [err_pos_4]
  cal err_pos_i agent 5/1(err_pos_5) -> [err_pos_5]
  [ksi_i_vec] -> cal err_pos_i agent 5/2(ksi_i_vec)
  [ksi_ld_hat_vec] -> cal err_pos_i agent 5/3(ksi_ld_hat_vec)
  [err_pos_5] -> combine err_pos_i/5(err_pos_5)
  [err_pos_3] -> combine err_pos_i/3(err_pos_3)
  [err_pos_4] -> combine err_pos_i/4(err_pos_4)
  [err_pos_2] -> combine err_pos_i/2(err_pos_2)
  [err_pos_1] -> combine err_pos_i/1(err_pos_1)
  combine err_pos_i/1(err_pos_vec) -> [err_pos_vec]
  cal err_vel_i agent 1/1(err_vel_1) -> [err_vel_1]
  [eta_i_vec] -> cal err_vel_i agent 1/2(eta_i_vec)
  [eta_ld_hat_vec] -> cal err_vel_i agent 1/3(eta_ld_hat_vec)
  [eta_ld_hat_vec] -> cal err_vel_i agent 2/3(eta_ld_hat_vec)
  cal err_vel_i agent 2/1(err_vel_2) -> [err_vel_2]
  [eta_i_vec] -> cal err_vel_i agent 2/2(eta_i_vec)
  [eta_i_vec] -> cal err_vel_i agent 3/2(eta_i_vec)
  cal err_vel_i agent 3/1(err_vel_3) -> [err_vel_3]
  [eta_ld_hat_vec] -> cal err_vel_i agent 3/3(eta_ld_hat_vec)
  [eta_ld_hat_vec] -> cal err_vel_i agent 4/3(eta_ld_hat_vec)
  cal err_vel_i agent 4/1(err_vel_4) -> [err_vel_4]
  [eta_i_vec] -> cal err_vel_i agent 4/2(eta_i_vec)
  [eta_i_vec] -> cal err_vel_i agent 5/2(eta_i_vec)
  cal err_vel_i agent 5/1(err_vel_5) -> [err_vel_5]
  [eta_ld_hat_vec] -> cal err_vel_i agent 5/3(eta_ld_hat_vec)
  [err_vel_2] -> combine err_vel_i/2(err_vel_2)
  [err_vel_3] -> combine err_vel_i/3(err_vel_3)
  [err_vel_4] -> combine err_vel_i/4(err_vel_4)
  [err_vel_1] -> combine err_vel_i/1(err_vel_1)
  combine err_vel_i/1(err_vel_vec) -> [err_vel_vec]
  [err_vel_5] -> combine err_vel_i/5(err_vel_5)
  [err_pos_vec] -> cal err_pos_bar_i agent 1/1(err_pos_vec)
  [phi_vec] -> cal err_pos_bar_i agent 1/2(phi_vec)
  cal err_pos_bar_i agent 1/1(err_pos_bar_1) -> [err_pos_bar_1]
  cal err_pos_bar_i agent 2/1(err_pos_bar_2) -> [err_pos_bar_2]
  [phi_vec] -> cal err_pos_bar_i agent 2/2(phi_vec)
  [err_pos_vec] -> cal err_pos_bar_i agent 2/1(err_pos_vec)
  cal err_pos_bar_i agent 3/1(err_pos_bar_3) -> [err_pos_bar_3]
  [phi_vec] -> cal err_pos_bar_i agent 3/2(phi_vec)
  [err_pos_vec] -> cal err_pos_bar_i agent 3/1(err_pos_vec)
  cal err_pos_bar_i agent 4/1(err_pos_bar_4) -> [err_pos_bar_4]
  [phi_vec] -> cal err_pos_bar_i agent 4/2(phi_vec)
  [err_pos_vec] -> cal err_pos_bar_i agent 4/1(err_pos_vec)
  [err_pos_vec] -> cal err_pos_bar_i agent 5/1(err_pos_vec)
  [phi_vec] -> cal err_pos_bar_i agent 5/2(phi_vec)
  cal err_pos_bar_i agent 5/1(err_pos_bar_5) -> [err_pos_bar_5]
  [err_pos_bar_5] -> combine err_pos_bar_i/5(err_pos_bar_5)
  combine err_pos_bar_i/1(err_pos_bar_vec) -> [err_pos_bar_vec]
  [err_pos_bar_1] -> combine err_pos_bar_i/1(err_pos_bar_1)
  [err_pos_bar_2] -> combine err_pos_bar_i/2(err_pos_bar_2)
  [err_pos_bar_4] -> combine err_pos_bar_i/4(err_pos_bar_4)
  [err_pos_bar_3] -> combine err_pos_bar_i/3(err_pos_bar_3)
  cal err_vel_bar_i agent 1/1(err_vel_bar_1) -> [err_vel_bar_1]
  [d_phi_vec] -> cal err_vel_bar_i agent 1/2(d_phi_vec)
  [err_vel_vec] -> cal err_vel_bar_i agent 1/1(err_vel_vec)
  [d_phi_vec] -> cal err_vel_bar_i agent 2/2(d_phi_vec)
  [err_vel_vec] -> cal err_vel_bar_i agent 2/1(err_vel_vec)
  cal err_vel_bar_i agent 2/1(err_vel_bar_2) -> [err_vel_bar_2]
  cal err_vel_bar_i agent 3/1(err_vel_bar_3) -> [err_vel_bar_3]
  [err_vel_vec] -> cal err_vel_bar_i agent 3/1(err_vel_vec)
  [d_phi_vec] -> cal err_vel_bar_i agent 3/2(d_phi_vec)
  cal err_vel_bar_i agent 4/1(err_vel_bar_4) -> [err_vel_bar_4]
  [err_vel_vec] -> cal err_vel_bar_i agent 4/1(err_vel_vec)
  [d_phi_vec] -> cal err_vel_bar_i agent 4/2(d_phi_vec)
  cal err_vel_bar_i agent 5/1(err_vel_bar_5) -> [err_vel_bar_5]
  [err_vel_vec] -> cal err_vel_bar_i agent 5/1(err_vel_vec)
  [d_phi_vec] -> cal err_vel_bar_i agent 5/2(d_phi_vec)
  [err_vel_bar_3] -> combine err_vel_bar/3(err_vel_bar_3)
  [err_vel_bar_4] -> combine err_vel_bar/4(err_vel_bar_4)
  [err_vel_bar_2] -> combine err_vel_bar/2(err_vel_bar_2)
  [err_vel_bar_1] -> combine err_vel_bar/1(err_vel_bar_1)
  combine err_vel_bar/1(err_vel_bar_vec) -> [err_vel_bar_vec]
  [err_vel_bar_5] -> combine err_vel_bar/5(err_vel_bar_5)
  [ksi_i_vec] -> cal pos_bar_i agent 1/1(ksi_i_vec)
  [phi_vec] -> cal pos_bar_i agent 1/2(phi_vec)
  cal pos_bar_i agent 1/1(pos_bar_1) -> [pos_bar_1]
  cal pos_bar_i agent 2/1(pos_bar_2) -> [pos_bar_2]
  [ksi_i_vec] -> cal pos_bar_i agent 2/1(ksi_i_vec)
  [phi_vec] -> cal pos_bar_i agent 2/2(phi_vec)
  [ksi_i_vec] -> cal pos_bar_i agent 3/1(ksi_i_vec)
  [phi_vec] -> cal pos_bar_i agent 3/2(phi_vec)
  cal pos_bar_i agent 3/1(pos_bar_3) -> [pos_bar_3]
  [ksi_i_vec] -> cal pos_bar_i agent 4/1(ksi_i_vec)
  [phi_vec] -> cal pos_bar_i agent 4/2(phi_vec)
  cal pos_bar_i agent 4/1(pos_bar_4) -> [pos_bar_4]
  cal pos_bar_i agent 5/1(pos_bar_5) -> [pos_bar_5]
  [ksi_i_vec] -> cal pos_bar_i agent 5/1(ksi_i_vec)
  [phi_vec] -> cal pos_bar_i agent 5/2(phi_vec)
  [pos_bar_5] -> combine pos_bar_i/5(pos_bar_5)
  [pos_bar_4] -> combine pos_bar_i/4(pos_bar_4)
  [pos_bar_1] -> combine pos_bar_i/1(pos_bar_1)
  [pos_bar_3] -> combine pos_bar_i/3(pos_bar_3)
  [pos_bar_2] -> combine pos_bar_i/2(pos_bar_2)
  Constant50/1 -> update event trigger state agent 1/1(c0)
  Constant52/1 -> update event trigger state agent 1/2(alfa)
  [tsim] -> update event trigger state agent 1/3(tsim)
  [pos_bar_vec] -> update event trigger state agent 1/4(pos_bar_vec)
  [ksi_ld_hat_vec] -> update event trigger state agent 1/5(ksi_ld_hat_vec)
  [pos_bar_tk_vec] -> update event trigger state agent 1/7(pos_bar_tk_vec)
  [ksi_ld_hat_tk_vec] -> update event trigger state agent 1/8(ksi_ld_hat_tk_vec)
  update event trigger state agent 1/2(pos_bar_tk_1) -> [pos_bar_tk_1]
  update event trigger state agent 1/3(ksi_ld_hat_tk_1) -> [ksi_ld_hat_tk_1]
  [tk_vec] -> update event trigger state agent 1/6(tk_vec)
  update event trigger state agent 1/1(tk_1) -> [tk_1]
  [ksi_ld_hat_tk_vec] -> update event trigger state agent 2/8(ksi_ld_hat_tk_vec)
  [tsim] -> update event trigger state agent 2/3(tsim)
  [ksi_ld_hat_vec] -> update event trigger state agent 2/5(ksi_ld_hat_vec)
  update event trigger state agent 2/2(pos_bar_tk_2) -> [pos_bar_tk_2]
  [pos_bar_tk_vec] -> update event trigger state agent 2/7(pos_bar_tk_vec)
  update event trigger state agent 2/3(ksi_ld_hat_tk_2) -> [ksi_ld_hat_tk_2]
  Constant54/1 -> update event trigger state agent 2/2(alfa)
  [pos_bar_vec] -> update event trigger state agent 2/4(pos_bar_vec)
  [tk_vec] -> update event trigger state agent 2/6(tk_vec)
  update event trigger state agent 2/1(tk_2) -> [tk_2]
  Constant53/1 -> update event trigger state agent 2/1(c0)
  Constant55/1 -> update event trigger state agent 3/1(c0)
  [tk_vec] -> update event trigger state agent 3/6(tk_vec)
  update event trigger state agent 3/3(ksi_ld_hat_tk_3) -> [ksi_ld_hat_tk_3]
  Constant56/1 -> update event trigger state agent 3/2(alfa)
  update event trigger state agent 3/2(pos_bar_tk_3) -> [pos_bar_tk_3]
  [pos_bar_tk_vec] -> update event trigger state agent 3/7(pos_bar_tk_vec)
  [ksi_ld_hat_vec] -> update event trigger state agent 3/5(ksi_ld_hat_vec)
  update event trigger state agent 3/1(tk_3) -> [tk_3]
  [tsim] -> update event trigger state agent 3/3(tsim)
  [pos_bar_vec] -> update event trigger state agent 3/4(pos_bar_vec)
  [ksi_ld_hat_tk_vec] -> update event trigger state agent 3/8(ksi_ld_hat_tk_vec)
  [ksi_ld_hat_tk_vec] -> update event trigger state agent 4/8(ksi_ld_hat_tk_vec)
  [tsim] -> update event trigger state agent 4/3(tsim)
  [ksi_ld_hat_vec] -> update event trigger state agent 4/5(ksi_ld_hat_vec)
  update event trigger state agent 4/1(tk_4) -> [tk_4]
  update event trigger state agent 4/3(ksi_ld_hat_tk_4) -> [ksi_ld_hat_tk_4]
  [tk_vec] -> update event trigger state agent 4/6(tk_vec)
  update event trigger state agent 4/2(pos_bar_tk_4) -> [pos_bar_tk_4]
  Constant58/1 -> update event trigger state agent 4/2(alfa)
  [pos_bar_vec] -> update event trigger state agent 4/4(pos_bar_vec)
  Constant57/1 -> update event trigger state agent 4/1(c0)
  [pos_bar_tk_vec] -> update event trigger state agent 4/7(pos_bar_tk_vec)
  Constant59/1 -> update event trigger state agent 5/1(c0)
  [pos_bar_tk_vec] -> update event trigger state agent 5/7(pos_bar_tk_vec)
  [ksi_ld_hat_vec] -> update event trigger state agent 5/5(ksi_ld_hat_vec)
  [pos_bar_vec] -> update event trigger state agent 5/4(pos_bar_vec)
  update event trigger state agent 5/2(pos_bar_tk_5) -> [pos_bar_tk_5]
  update event trigger state agent 5/1(tk_5) -> [tk_5]
  [tk_vec] -> update event trigger state agent 5/6(tk_vec)
  [tsim] -> update event trigger state agent 5/3(tsim)
  Constant60/1 -> update event trigger state agent 5/2(alfa)
  [ksi_ld_hat_tk_vec] -> update event trigger state agent 5/8(ksi_ld_hat_tk_vec)
  update event trigger state agent 5/3(ksi_ld_hat_tk_5) -> [ksi_ld_hat_tk_5]
  combine event trigger tk/1(tk_vec) -> Memory9/1
  [tk_5] -> combine event trigger tk/5(tk_5)
  [tk_4] -> combine event trigger tk/4(tk_4)
  Memory9/1 -> [tk_vec]
  [tk_3] -> combine event trigger tk/3(tk_3)
  [tk_1] -> combine event trigger tk/1(tk_1)
  [tk_2] -> combine event trigger tk/2(tk_2)
  [pos_bar_tk_5] -> combine event trigger pos_bar_tk/5(pos_bar_tk_5)
  Memory10/1 -> [pos_bar_tk_vec]
  combine event trigger pos_bar_tk/1(pos_bar_tk_vec) -> Memory10/1
  [pos_bar_tk_2] -> combine event trigger pos_bar_tk/2(pos_bar_tk_2)
  [pos_bar_tk_1] -> combine event trigger pos_bar_tk/1(pos_bar_tk_1)
  [pos_bar_tk_4] -> combine event trigger pos_bar_tk/4(pos_bar_tk_4)
  [pos_bar_tk_3] -> combine event trigger pos_bar_tk/3(pos_bar_tk_3)
  [ksi_ld_hat_tk_2] -> combine event trigger ksi_ld_hat_tk/2(ksi_ld_hat_tk_2)
  [ksi_ld_hat_tk_1] -> combine event trigger ksi_ld_hat_tk/1(ksi_ld_hat_tk_1)
  combine event trigger ksi_ld_hat_tk/1(ksi_ld_hat_tk_vec) -> Memory11/1
  [ksi_ld_hat_tk_3] -> combine event trigger ksi_ld_hat_tk/3(ksi_ld_hat_tk_3)
  [ksi_ld_hat_tk_4] -> combine event trigger ksi_ld_hat_tk/4(ksi_ld_hat_tk_4)
  [ksi_ld_hat_tk_5] -> combine event trigger ksi_ld_hat_tk/5(ksi_ld_hat_tk_5)
  Memory11/1 -> [ksi_ld_hat_tk_vec]
  Constant61/1 -> cal Di agent 1/1(Wij)
  [pos_bar_tk_vec] -> cal Di agent 1/3(pos_bar_tk_vec)
  [ksi_ld_hat_tk_vec] -> cal Di agent 1/4(ksi_ld_hat_tk_vec)
  [ksi_ld_hat_vec] -> cal Di agent 1/5(ksi_ld_hat_vec)
  cal Di agent 1/1(Di_1) -> [Di_1]
  cal Di agent 2/1(Di_2) -> [Di_2]
  [ksi_ld_hat_tk_vec] -> cal Di agent 2/4(ksi_ld_hat_tk_vec)
  Constant63/1 -> cal Di agent 2/1(Wij)
  [pos_bar_tk_vec] -> cal Di agent 2/3(pos_bar_tk_vec)
  [ksi_ld_hat_vec] -> cal Di agent 2/5(ksi_ld_hat_vec)
  Constant65/1 -> cal Di agent 3/1(Wij)
  [pos_bar_tk_vec] -> cal Di agent 3/3(pos_bar_tk_vec)
  [ksi_ld_hat_vec] -> cal Di agent 3/5(ksi_ld_hat_vec)
  [ksi_ld_hat_tk_vec] -> cal Di agent 3/4(ksi_ld_hat_tk_vec)
  cal Di agent 3/1(Di_3) -> [Di_3]
  [ksi_ld_hat_vec] -> cal Di agent 4/5(ksi_ld_hat_vec)
  Constant67/1 -> cal Di agent 4/1(Wij)
  [ksi_ld_hat_tk_vec] -> cal Di agent 4/4(ksi_ld_hat_tk_vec)
  [pos_bar_tk_vec] -> cal Di agent 4/3(pos_bar_tk_vec)
  cal Di agent 4/1(Di_4) -> [Di_4]
  [pos_bar_tk_vec] -> cal Di agent 5/3(pos_bar_tk_vec)
  cal Di agent 5/1(Di_5) -> [Di_5]
  Constant69/1 -> cal Di agent 5/1(Wij)
  [ksi_ld_hat_vec] -> cal Di agent 5/5(ksi_ld_hat_vec)
  [ksi_ld_hat_tk_vec] -> cal Di agent 5/4(ksi_ld_hat_tk_vec)
  combine Di_vec/1(Di_vec) -> Memory12/1
  [Di_5] -> combine Di_vec/5(Di_5)
  [Di_4] -> combine Di_vec/4(Di_4)
  Memory12/1 -> [Di_vec]
  [Di_3] -> combine Di_vec/3(Di_3)
  [Di_1] -> combine Di_vec/1(Di_1)
  [Di_2] -> combine Di_vec/2(Di_2)
  Constant71/1 -> cal x4i agent 1/1(Wij)
  Constant72/1 -> cal x4i agent 1/2(lam4)
  [x4i_vec] -> cal x4i agent 1/3(x4i_vec)
  [Di_vec] -> cal x4i agent 1/4(Di_vec)
  [eta_ld_hat_vec] -> cal x4i agent 1/5(eta_ld_hat_vec)
  cal x4i agent 1/1(d_x4i_1) -> x4i Integrator agent 1/1
  x4i Integrator agent 1/1 -> [x4i_1]
  cal x4i agent 2/1(d_x4i_2) -> x4i Integrator agent 2/1
  Constant73/1 -> cal x4i agent 2/1(Wij)
  x4i Integrator agent 2/1 -> [x4i_2]
  [x4i_vec] -> cal x4i agent 2/3(x4i_vec)
  [eta_ld_hat_vec] -> cal x4i agent 2/5(eta_ld_hat_vec)
  Constant74/1 -> cal x4i agent 2/2(lam4)
  [Di_vec] -> cal x4i agent 2/4(Di_vec)
  Constant76/1 -> cal x4i agent 3/2(lam4)
  [Di_vec] -> cal x4i agent 3/4(Di_vec)
  [x4i_vec] -> cal x4i agent 3/3(x4i_vec)
  cal x4i agent 3/1(d_x4i_3) -> x4i Integrator agent 3/1
  x4i Integrator agent 3/1 -> [x4i_3]
  Constant75/1 -> cal x4i agent 3/1(Wij)
  [eta_ld_hat_vec] -> cal x4i agent 3/5(eta_ld_hat_vec)
  cal x4i agent 4/1(d_x4i_4) -> x4i Integrator agent 4/1
  x4i Integrator agent 4/1 -> [x4i_4]
  Constant77/1 -> cal x4i agent 4/1(Wij)
  [eta_ld_hat_vec] -> cal x4i agent 4/5(eta_ld_hat_vec)
  [Di_vec] -> cal x4i agent 4/4(Di_vec)
  Constant78/1 -> cal x4i agent 4/2(lam4)
  [x4i_vec] -> cal x4i agent 4/3(x4i_vec)
  Constant80/1 -> cal x4i agent 5/2(lam4)
  [Di_vec] -> cal x4i agent 5/4(Di_vec)
  [x4i_vec] -> cal x4i agent 5/3(x4i_vec)
  [eta_ld_hat_vec] -> cal x4i agent 5/5(eta_ld_hat_vec)
  cal x4i agent 5/1(d_x4i_5) -> x4i Integrator agent 5/1
  Constant79/1 -> cal x4i agent 5/1(Wij)
  x4i Integrator agent 5/1 -> [x4i_5]
  [x4i_1] -> combine x4i/1(x4i_1)
  [x4i_2] -> combine x4i/2(x4i_2)
  combine x4i/1(x4i_vec) -> Memory13/1
  [x4i_5] -> combine x4i/5(x4i_5)
  [x4i_3] -> combine x4i/3(x4i_3)
  Memory13/1 -> [x4i_vec]
  [x4i_4] -> combine x4i/4(x4i_4)
  cal x3i agent 1/1(d_x3i_1) -> x3i Integrator agent 1/1
  x3i Integrator agent 1/1 -> [x3i_1]
  Constant82/1 -> cal x3i agent 1/1(lam3)
  [x3i_vec] -> cal x3i agent 1/2(x3i_vec)
  [x4i_vec] -> cal x3i agent 1/3(x4i_vec)
  [eta_ld_hat_vec] -> cal x3i agent 1/4(eta_ld_hat_vec)
  Constant81/1 -> cal x3i agent 2/1(lam3)
  [eta_ld_hat_vec] -> cal x3i agent 2/4(eta_ld_hat_vec)
  [x3i_vec] -> cal x3i agent 2/2(x3i_vec)
  x3i Integrator agent 2/1 -> [x3i_2]
  [x4i_vec] -> cal x3i agent 2/3(x4i_vec)
  cal x3i agent 2/1(d_x3i_2) -> x3i Integrator agent 2/1
  x3i Integrator agent 3/1 -> [x3i_3]
  [x4i_vec] -> cal x3i agent 3/3(x4i_vec)
  Constant83/1 -> cal x3i agent 3/1(lam3)
  cal x3i agent 3/1(d_x3i_3) -> x3i Integrator agent 3/1
  [x3i_vec] -> cal x3i agent 3/2(x3i_vec)
  [eta_ld_hat_vec] -> cal x3i agent 3/4(eta_ld_hat_vec)
  cal x3i agent 4/1(d_x3i_4) -> x3i Integrator agent 4/1
  Constant84/1 -> cal x3i agent 4/1(lam3)
  x3i Integrator agent 4/1 -> [x3i_4]
  [x4i_vec] -> cal x3i agent 4/3(x4i_vec)
  [x3i_vec] -> cal x3i agent 4/2(x3i_vec)
  [eta_ld_hat_vec] -> cal x3i agent 4/4(eta_ld_hat_vec)
  x3i Integrator agent 5/1 -> [x3i_5]
  [x3i_vec] -> cal x3i agent 5/2(x3i_vec)
  cal x3i agent 5/1(d_x3i_5) -> x3i Integrator agent 5/1
  [x4i_vec] -> cal x3i agent 5/3(x4i_vec)
  [eta_ld_hat_vec] -> cal x3i agent 5/4(eta_ld_hat_vec)
  Constant85/1 -> cal x3i agent 5/1(lam3)
  [x3i_3] -> combine x3i/3(x3i_3)
  Memory14/1 -> [x3i_vec]
  [x3i_2] -> combine x3i/2(x3i_2)
  combine x3i/1(x3i_vec) -> Memory14/1
  [x3i_5] -> combine x3i/5(x3i_5)
  [x3i_4] -> combine x3i/4(x3i_4)
  [x3i_1] -> combine x3i/1(x3i_1)
  Constant86/1 -> cal x2i agent 1/1(lam2)
  [eta_ld_hat_vec] -> cal x2i agent 1/4(eta_ld_hat_vec)
  x2i Integrator agent 1/1 -> [x2i_1]
  cal x2i agent 1/1(d_x2i_1) -> x2i Integrator agent 1/1
  [x2i_vec] -> cal x2i agent 1/2(x2i_vec)
  [x3i_vec] -> cal x2i agent 1/3(x3i_vec)
  [x3i_vec] -> cal x2i agent 2/3(x3i_vec)
  cal x2i agent 2/1(d_x2i_2) -> x2i Integrator agent 2/1
  Constant87/1 -> cal x2i agent 2/1(lam2)
  [eta_ld_hat_vec] -> cal x2i agent 2/4(eta_ld_hat_vec)
  [x2i_vec] -> cal x2i agent 2/2(x2i_vec)
  x2i Integrator agent 2/1 -> [x2i_2]
  x2i Integrator agent 3/1 -> [x2i_3]
  [x2i_vec] -> cal x2i agent 3/2(x2i_vec)
  cal x2i agent 3/1(d_x2i_3) -> x2i Integrator agent 3/1
  [x3i_vec] -> cal x2i agent 3/3(x3i_vec)
  [eta_ld_hat_vec] -> cal x2i agent 3/4(eta_ld_hat_vec)
  Constant88/1 -> cal x2i agent 3/1(lam2)
  [x2i_vec] -> cal x2i agent 4/2(x2i_vec)
  x2i Integrator agent 4/1 -> [x2i_4]
  [x3i_vec] -> cal x2i agent 4/3(x3i_vec)
  Constant89/1 -> cal x2i agent 4/1(lam2)
  [eta_ld_hat_vec] -> cal x2i agent 4/4(eta_ld_hat_vec)
  cal x2i agent 4/1(d_x2i_4) -> x2i Integrator agent 4/1
  [eta_ld_hat_vec] -> cal x2i agent 5/4(eta_ld_hat_vec)
  [x3i_vec] -> cal x2i agent 5/3(x3i_vec)
  x2i Integrator agent 5/1 -> [x2i_5]
  cal x2i agent 5/1(d_x2i_5) -> x2i Integrator agent 5/1
  Constant90/1 -> cal x2i agent 5/1(lam2)
  [x2i_vec] -> cal x2i agent 5/2(x2i_vec)
  [x2i_1] -> combine x2i/1(x2i_1)
  [x2i_2] -> combine x2i/2(x2i_2)
  combine x2i/1(x2i_vec) -> Memory15/1
  Memory15/1 -> [x2i_vec]
  [x2i_5] -> combine x2i/5(x2i_5)
  [x2i_3] -> combine x2i/3(x2i_3)
  [x2i_4] -> combine x2i/4(x2i_4)
  cal x1i agent 1/1(d_x1i_1) -> [d_x1i_1], x1i Integrator agent 1/1
  Constant91/1 -> cal x1i agent 1/1(lam1)
  [eta_ld_hat_vec] -> cal x1i agent 1/4(eta_ld_hat_vec)
  x1i Integrator agent 1/1 -> [x1i_1]
  [x1i_vec] -> cal x1i agent 1/2(x1i_vec)
  [x2i_vec] -> cal x1i agent 1/3(x2i_vec)
  cal x1i agent 2/1(d_x1i_2) -> [d_x1i_2], x1i Integrator agent 2/1
  Constant147/1 -> cal x1i agent 2/1(lam1)
  [x1i_vec] -> cal x1i agent 2/2(x1i_vec)
  x1i Integrator agent 2/1 -> [x1i_2]
  [eta_ld_hat_vec] -> cal x1i agent 2/4(eta_ld_hat_vec)
  [x2i_vec] -> cal x1i agent 2/3(x2i_vec)
  [x1i_vec] -> cal x1i agent 3/2(x1i_vec)
  x1i Integrator agent 3/1 -> [x1i_3]
  Constant148/1 -> cal x1i agent 3/1(lam1)
  [eta_ld_hat_vec] -> cal x1i agent 3/4(eta_ld_hat_vec)
  [x2i_vec] -> cal x1i agent 3/3(x2i_vec)
  cal x1i agent 3/1(d_x1i_3) -> [d_x1i_3], x1i Integrator agent 3/1
  x1i Integrator agent 4/1 -> [x1i_4]
  [x1i_vec] -> cal x1i agent 4/2(x1i_vec)
  cal x1i agent 4/1(d_x1i_4) -> [d_x1i_4], x1i Integrator agent 4/1
  [eta_ld_hat_vec] -> cal x1i agent 4/4(eta_ld_hat_vec)
  [x2i_vec] -> cal x1i agent 4/3(x2i_vec)
  Constant149/1 -> cal x1i agent 4/1(lam1)
  Constant150/1 -> cal x1i agent 5/1(lam1)
  [eta_ld_hat_vec] -> cal x1i agent 5/4(eta_ld_hat_vec)
  [x2i_vec] -> cal x1i agent 5/3(x2i_vec)
  x1i Integrator agent 5/1 -> [x1i_5]
  [x1i_vec] -> cal x1i agent 5/2(x1i_vec)
  cal x1i agent 5/1(d_x1i_5) -> [d_x1i_5], x1i Integrator agent 5/1
  [x1i_3] -> combine x1i/3(x1i_3)
  [x1i_4] -> combine x1i/4(x1i_4)
  [x1i_5] -> combine x1i/5(x1i_5)
  Memory16/1 -> [x1i_vec]
  [x1i_2] -> combine x1i/2(x1i_2)
  combine x1i/1(x1i_vec) -> Memory16/1
  [x1i_1] -> combine x1i/1(x1i_1)
  [x1i_vec] -> cal yi/1(x1i_vec)
  cal yi/1(yi_vec) -> [yi_vec]
  Constant151/1 -> cal betai agent 1/1(gamma0)
  [pos_bar_vec] -> cal betai agent 1/2(pos_bar_vec)
  [yi_vec] -> cal betai agent 1/3(yi_vec)
  cal betai agent 1/1(betai_1) -> [beta_1]
  [yi_vec] -> cal betai agent 2/3(yi_vec)
  cal betai agent 2/1(betai_2) -> [beta_2]
  Constant152/1 -> cal betai agent 2/1(gamma0)
  [pos_bar_vec] -> cal betai agent 2/2(pos_bar_vec)
  cal betai agent 3/1(betai_3) -> [beta_3]
  [pos_bar_vec] -> cal betai agent 3/2(pos_bar_vec)
  Constant153/1 -> cal betai agent 3/1(gamma0)
  [yi_vec] -> cal betai agent 3/3(yi_vec)
  [pos_bar_vec] -> cal betai agent 4/2(pos_bar_vec)
  Constant154/1 -> cal betai agent 4/1(gamma0)
  [yi_vec] -> cal betai agent 4/3(yi_vec)
  cal betai agent 4/1(betai_4) -> [beta_4]
  [yi_vec] -> cal betai agent 5/3(yi_vec)
  Constant155/1 -> cal betai agent 5/1(gamma0)
  [pos_bar_vec] -> cal betai agent 5/2(pos_bar_vec)
  cal betai agent 5/1(betai_5) -> [beta_5]
  combine beta/1(beta_vec) -> Memory17/1
  Memory17/1 -> [beta_vec]
  [beta_4] -> combine beta/4(beta_4)
  [beta_3] -> combine beta/3(beta_3)
  [beta_5] -> combine beta/5(beta_5)
  [beta_1] -> combine beta/1(beta_1)
  [beta_2] -> combine beta/2(beta_2)
  combine d_xi1/1(d_x1i_vec) -> Memory18/1
  Memory18/1 -> [d_x1i_vec]
  [d_x1i_4] -> combine d_xi1/4(d_x1i_4)
  [d_x1i_3] -> combine d_xi1/3(d_x1i_3)
  [d_x1i_5] -> combine d_xi1/5(d_x1i_5)
  [d_x1i_1] -> combine d_xi1/1(d_x1i_1)
  [d_x1i_2] -> combine d_xi1/2(d_x1i_2)
  cal d_yi/1(d_yi_vec) -> [d_yi_vec]
  [d_x1i_vec] -> cal d_yi/1(d_x1i_vec)
  Constant156/1 -> cal d_betai agent 1/1(gamma0)
  [eta_i_vec] -> cal d_betai agent 1/2(eta_i_vec)
  [d_phi_vec] -> cal d_betai agent 1/3(d_phi_vec)
  [d_yi_vec] -> cal d_betai agent 1/4(d_yi_vec)
  cal d_betai agent 1/1(d_betai_1) -> [d_betai_1]
  cal d_betai agent 2/1(d_betai_2) -> [d_betai_2]
  Constant157/1 -> cal d_betai agent 2/1(gamma0)
  [d_yi_vec] -> cal d_betai agent 2/4(d_yi_vec)
  [d_phi_vec] -> cal d_betai agent 2/3(d_phi_vec)
  [eta_i_vec] -> cal d_betai agent 2/2(eta_i_vec)
  Constant158/1 -> cal d_betai agent 3/1(gamma0)
  [d_yi_vec] -> cal d_betai agent 3/4(d_yi_vec)
  cal d_betai agent 3/1(d_betai_3) -> [d_betai_3]
  [d_phi_vec] -> cal d_betai agent 3/3(d_phi_vec)
  [eta_i_vec] -> cal d_betai agent 3/2(eta_i_vec)
  [d_phi_vec] -> cal d_betai agent 4/3(d_phi_vec)
  [eta_i_vec] -> cal d_betai agent 4/2(eta_i_vec)
  cal d_betai agent 4/1(d_betai_4) -> [d_betai_4]
  Constant159/1 -> cal d_betai agent 4/1(gamma0)
  [d_yi_vec] -> cal d_betai agent 4/4(d_yi_vec)
  Constant160/1 -> cal d_betai agent 5/1(gamma0)
  cal d_betai agent 5/1(d_betai_5) -> [d_betai_5]
  [eta_i_vec] -> cal d_betai agent 5/2(eta_i_vec)
  [d_yi_vec] -> cal d_betai agent 5/4(d_yi_vec)
  [d_phi_vec] -> cal d_betai agent 5/3(d_phi_vec)
  [d_betai_5] -> combine d_betai/5(d_beta_5)
  [d_betai_1] -> combine d_betai/1(d_beta_1)
  [d_betai_2] -> combine d_betai/2(d_beta_2)
  Memory19/1 -> [d_beta_vec]
  [d_betai_4] -> combine d_betai/4(d_beta_4)
  combine d_betai/1(d_beta_vec) -> Memory19/1
  [d_betai_3] -> combine d_betai/3(d_beta_3)
  Constant162/1 -> cal thetai agent 1/1(k_theta)
  [err_vel_vec] -> cal thetai agent 1/2(err_vel_vec)
  [beta_vec] -> cal thetai agent 1/3(beta_vec)
  [d_beta_vec] -> cal thetai agent 1/4(d_beta_vec)
  cal thetai agent 1/1(thetai_1) -> [theta_1]
  Constant163/1 -> cal thetai agent 2/1(k_theta)
  [d_beta_vec] -> cal thetai agent 2/4(d_beta_vec)
  [beta_vec] -> cal thetai agent 2/3(beta_vec)
  cal thetai agent 2/1(thetai_2) -> [theta_2]
  [err_vel_vec] -> cal thetai agent 2/2(err_vel_vec)
  [err_vel_vec] -> cal thetai agent 3/2(err_vel_vec)
  [d_beta_vec] -> cal thetai agent 3/4(d_beta_vec)
  cal thetai agent 3/1(thetai_3) -> [theta_3]
  [beta_vec] -> cal thetai agent 3/3(beta_vec)
  Constant164/1 -> cal thetai agent 3/1(k_theta)
  cal thetai agent 4/1(thetai_4) -> [theta_4]
  [beta_vec] -> cal thetai agent 4/3(beta_vec)
  [err_vel_vec] -> cal thetai agent 4/2(err_vel_vec)
  Constant165/1 -> cal thetai agent 4/1(k_theta)
  [d_beta_vec] -> cal thetai agent 4/4(d_beta_vec)
  Constant166/1 -> cal thetai agent 5/1(k_theta)
  [err_vel_vec] -> cal thetai agent 5/2(err_vel_vec)
  cal thetai agent 5/1(thetai_5) -> [theta_5]
  [beta_vec] -> cal thetai agent 5/3(beta_vec)
  [d_beta_vec] -> cal thetai agent 5/4(d_beta_vec)
  combine thetai/1(theta_vec) -> Memory20/1
  [theta_3] -> combine thetai/3(theta_3)
  [theta_2] -> combine thetai/2(theta_2)
  Memory20/1 -> [theta_vec]
  [theta_4] -> combine thetai/4(theta_4)
  [theta_1] -> combine thetai/1(theta_1)
  [theta_5] -> combine thetai/5(theta_5)
  Constant167/1 -> cal phi agent 1/1(k_phi)
  [phi_vec] -> cal phi agent 1/2(phi_vec)
  [d_phi_vec] -> cal phi agent 1/3(d_phi_vec)
  [theta_vec] -> cal phi agent 1/4(theta_vec)
  cal phi agent 1/1(d2_phi_1) -> d_phi Integrator agent 1/1
  d_phi Integrator agent 1/1 -> [d_phi_1], phi Integrator agent 1/1
  phi Integrator agent 1/1 -> [phi_1]
  d_phi Integrator agent 2/1 -> [d_phi_2], phi Integrator agent 2/1
  [d_phi_vec] -> cal phi agent 2/3(d_phi_vec)
  cal phi agent 2/1(d2_phi_2) -> d_phi Integrator agent 2/1
  [theta_vec] -> cal phi agent 2/4(theta_vec)
  phi Integrator agent 2/1 -> [phi_2]
  [phi_vec] -> cal phi agent 2/2(phi_vec)
  Constant168/1 -> cal phi agent 2/1(k_phi)
  Constant169/1 -> cal phi agent 3/1(k_phi)
  phi Integrator agent 3/1 -> [phi_3]
  cal phi agent 3/1(d2_phi_3) -> d_phi Integrator agent 3/1
  [phi_vec] -> cal phi agent 3/2(phi_vec)
  [d_phi_vec] -> cal phi agent 3/3(d_phi_vec)
  d_phi Integrator agent 3/1 -> [d_phi_3], phi Integrator agent 3/1
  [theta_vec] -> cal phi agent 3/4(theta_vec)
  [theta_vec] -> cal phi agent 4/4(theta_vec)
  [d_phi_vec] -> cal phi agent 4/3(d_phi_vec)
  d_phi Integrator agent 4/1 -> [d_phi_4], phi Integrator agent 4/1
  Constant170/1 -> cal phi agent 4/1(k_phi)
  cal phi agent 4/1(d2_phi_4) -> d_phi Integrator agent 4/1
  phi Integrator agent 4/1 -> [phi_4]
  [phi_vec] -> cal phi agent 4/2(phi_vec)
  phi Integrator agent 5/1 -> [phi_5]
  [phi_vec] -> cal phi agent 5/2(phi_vec)
  cal phi agent 5/1(d2_phi_5) -> d_phi Integrator agent 5/1
  [d_phi_vec] -> cal phi agent 5/3(d_phi_vec)
  d_phi Integrator agent 5/1 -> [d_phi_5], phi Integrator agent 5/1
  Constant171/1 -> cal phi agent 5/1(k_phi)
  [theta_vec] -> cal phi agent 5/4(theta_vec)
  [d_phi_5] -> combine d_phi/5(d_phi_5)
  [d_phi_2] -> combine d_phi/2(d_phi_2)
  [d_phi_4] -> combine d_phi/4(d_phi_4)
  [d_phi_1] -> combine d_phi/1(d_phi_1)
  [d_phi_3] -> combine d_phi/3(d_phi_3)
  combine d_phi/1(d_phi_vec) -> Memory21/1
  Memory21/1 -> [d_phi_vec]
  [phi_4] -> combine phi/4(phi_4)
  combine phi/1(phi_vec) -> Memory22/1
  [phi_1] -> combine phi/1(phi_1)
  [phi_3] -> combine phi/3(phi_3)
  [phi_2] -> combine phi/2(phi_2)
  Memory22/1 -> [phi_vec]
  [phi_5] -> combine phi/5(phi_5)
  Constant172/1 -> cal ui agent 1/1(k_phi)
  [rho_hat_vec] -> cal ui agent 1/2(rho_hat_vec)
  [phi_vec] -> cal ui agent 1/3(phi_vec)
  [d_phi_vec] -> cal ui agent 1/4(d_phi_vec)
  [dp_hat_vec] -> cal ui agent 1/5(dp_hat_vec)
  Constant173/1 -> cal ui agent 2/1(k_phi)
  [rho_hat_vec] -> cal ui agent 2/2(rho_hat_vec)
  [phi_vec] -> cal ui agent 2/3(phi_vec)
  [d_phi_vec] -> cal ui agent 2/4(d_phi_vec)
  [dp_hat_vec] -> cal ui agent 2/5(dp_hat_vec)
  Constant174/1 -> cal ui agent 3/1(k_phi)
  [rho_hat_vec] -> cal ui agent 3/2(rho_hat_vec)
  [phi_vec] -> cal ui agent 3/3(phi_vec)
  [d_phi_vec] -> cal ui agent 3/4(d_phi_vec)
  [dp_hat_vec] -> cal ui agent 3/5(dp_hat_vec)
  Constant175/1 -> cal ui agent 4/1(k_phi)
  [rho_hat_vec] -> cal ui agent 4/2(rho_hat_vec)
  [phi_vec] -> cal ui agent 4/3(phi_vec)
  [d_phi_vec] -> cal ui agent 4/4(d_phi_vec)
  [dp_hat_vec] -> cal ui agent 4/5(dp_hat_vec)
  Constant176/1 -> cal ui agent 5/1(k_phi)
  [rho_hat_vec] -> cal ui agent 5/2(rho_hat_vec)
  [phi_vec] -> cal ui agent 5/3(phi_vec)
  [d_phi_vec] -> cal ui agent 5/4(d_phi_vec)
  [dp_hat_vec] -> cal ui agent 5/5(dp_hat_vec)
  cal vel_bar_i agent 1/1(vel_bar_1) -> [vel_bar_1]
  [eta_i_vec] -> cal vel_bar_i agent 1/1(eta_i_vec)
  [phi_vec] -> cal vel_bar_i agent 1/2(d_phi_vec)
  [phi_vec] -> cal vel_bar_i agent 2/2(d_phi_vec)
  [eta_i_vec] -> cal vel_bar_i agent 2/1(eta_i_vec)
  cal vel_bar_i agent 2/1(vel_bar_2) -> [vel_bar_2]
  cal vel_bar_i agent 3/1(vel_bar_3) -> [vel_bar_3]
  [phi_vec] -> cal vel_bar_i agent 3/2(d_phi_vec)
  [eta_i_vec] -> cal vel_bar_i agent 3/1(eta_i_vec)
  [eta_i_vec] -> cal vel_bar_i agent 4/1(eta_i_vec)
  cal vel_bar_i agent 4/1(vel_bar_4) -> [vel_bar_4]
  [phi_vec] -> cal vel_bar_i agent 4/2(d_phi_vec)
  [phi_vec] -> cal vel_bar_i agent 5/2(d_phi_vec)
  [eta_i_vec] -> cal vel_bar_i agent 5/1(eta_i_vec)
  cal vel_bar_i agent 5/1(vel_bar_5) -> [vel_bar_5]
  [vel_bar_5] -> combine vel_bar_i/5(vel_bar_5)
  [vel_bar_4] -> combine vel_bar_i/4(vel_bar_4)
  [vel_bar_3] -> combine vel_bar_i/3(vel_bar_3)
  [vel_bar_1] -> combine vel_bar_i/1(vel_bar_1)
  [vel_bar_2] -> combine vel_bar_i/2(vel_bar_2)
  combine pos_bar_i/1(pos_bar_vec) -> Memory8/1
  combine vel_bar_i/1(vel_bar_vec) -> Memory23/1
  Memory8/1 -> [pos_bar_vec]
  Memory23/1 -> [vel_bar_vec]
  Constant180/1 -> process velocity/10(Rz2)
  Demux1/3 -> ksi_0/3
  [tsim] -> process velocity/11(t)
  Constant222/1 -> set desire formation configuration/8(Z2)
  leader eta0 Integrator/1 -> [eta0], leader ksi0 Integrator/1
  Constant185/1 -> set desire formation configuration/4(Y1)
  Constant188/1 -> leader control input/4(R0)
  [tsim] -> leader control input/1(t)
  Constant178/1 -> process velocity/7(R1)
  [ksi0] -> desire formation position and velocity/1(ksi0)
  Constant197/1 -> process velocity/5(PZ1)
  Constant235/1 -> set desire formation configuration/12(kai_3_t)
  [tsim] -> set desire formation configuration/15(t)
  process velocity/1(V_init_out) -> [V_init_out]
  Constant182/1 -> process velocity/8(Rx2)
  Constant184/1 -> set desire formation configuration/2(X2)
  Demux22/1 -> eta_0/1
  [delta_eta_vec] -> desire formation position and velocity/4(delta_eta_vec)
  Demux1/1 -> ksi_0/1
  Constant229/1 -> set desire formation configuration/6(Y3)
  Constant189/1 -> leader control input/5(R1)
  set desire formation configuration/1(delta_ksi_vec) -> [delta_ksi_vec]
  Constant195/1 -> process velocity/2(T1)
  desire formation position and velocity/2(vel_i_des) -> [vel_i_des]
  Constant221/1 -> set desire formation configuration/7(Z1)
  Constant177/1 -> process velocity/6(R0)
  Constant226/1 -> set desire formation configuration/9(Z3)
  Constant181/1 -> process velocity/9(Ry2)
  Demux22/3 -> eta_0/3
  Constant194/1 -> process velocity/3(T2)
  Demux1/2 -> ksi_0/2
  [ksi0] -> Demux1/1
  leader ksi0 Integrator/1 -> [ksi0]
  Constant234/1 -> set desire formation configuration/3(X3)
  Constant192/1 -> leader control input/7(Ry2)
  Constant161/1 -> leader control input/2(T1)
  Constant183/1 -> set desire formation configuration/1(X1)
  Constant193/1 -> leader control input/8(Rz2)
  [u0] -> leader eta0 Integrator/1
  Constant239/1 -> set desire formation configuration/14(T12)
  Demux22/2 -> eta_0/2
  Constant186/1 -> set desire formation configuration/5(Y2)
  Constant225/1 -> set desire formation configuration/10(theta0)
  Constant187/1 -> leader control input/3(T2)
  [eta0] -> Demux22/1
  Clock/1 -> [tsim]
  [V_init_out] -> leader eta0 Integrator/3
  Constant196/1 -> process velocity/4(PZ0)
  desire formation position and velocity/1(pos_i_des) -> [pos_i_des]
  Step/1 -> leader eta0 Integrator/2
  Constant231/1 -> set desire formation configuration/11(kai_1_t)
  [eta0] -> desire formation position and velocity/2(eta0)
  leader control input/1(u0) -> [u0]
  Constant238/1 -> set desire formation configuration/13(T1)
  Constant190/1 -> leader control input/6(Rx2)
  Constant179/1 -> process velocity/1(T0)
  set desire formation configuration/2(delta_eta_vec) -> [delta_eta_vec]
  [delta_ksi_vec] -> desire formation position and velocity/3(delta_ksi_vec)
  set desire formation configuration/3(d_delta_eta_vec) -> [d_delta_eta_vec]
  [eta_track_err_vec] -> To Workspace34/1
  [d_phi_vec] -> To Workspace32/1
  [pos_bar_tk_vec] -> To Workspace30/1
  [ksi_track_err_vec] -> To Workspace33/1
  [ksi_i_vec] -> To Workspace8/1
  [ksi_ld_hat_tk_vec] -> To Workspace29/1
  [d_yi_vec] -> To Workspace25/1
  [theta_vec] -> To Workspace28/1
  [phi_vec] -> To Workspace31/1
  [yi_vec] -> To Workspace23/1
  [sigma_v_vec] -> To Workspace19/1
  [u0] -> To Workspace3/1
  [err_pos_vec] -> To Workspace22/1
  [sigma_bar_v_tilt_vec] -> To Workspace13/1
  [sigma_bar_v_vec] -> To Workspace12/1
  [sigma_bar_v_hat_vec] -> To Workspace11/1
  [err_vel_bar_vec] -> To Workspace27/1
  [err_vel_vec] -> To Workspace21/1
  [dp_tilt_vec] -> To Workspace6/1
  [ui] -> To Workspace14/1
  [dp_hat_vec] -> To Workspace1/1
  [tk_vec] -> To Workspace18/1
  [rho_hat_vec] -> To Workspace17/1
  [eta_ld_hat_vec] -> To Workspace10/1
  [vel_bar_vec] -> To Workspace24/1
  [ksi_ld_hat_vec] -> To Workspace9/1
  [eta_i_vec] -> To Workspace7/1
  [err_pos_bar_vec] -> To Workspace26/1
  [ksi0] -> To Workspace5/1
  [pos_bar_vec] -> To Workspace16/1
  [beta_vec] -> To Workspace/1
  [d_beta_vec] -> To Workspace20/1
  [rho_err_vec] -> To Workspace15/1
  [dp_vec] -> To Workspace2/1
  [eta0] -> To Workspace4/1
  [delta_ksi_vec] -> cal err_pos_i agent 1/1(delta_ksi_vec)
  [delta_ksi_vec] -> cal err_pos_i agent 2/1(delta_ksi_vec)
  [delta_ksi_vec] -> cal err_pos_i agent 3/1(delta_ksi_vec)
  [delta_ksi_vec] -> cal err_pos_i agent 4/1(delta_ksi_vec)
  [delta_ksi_vec] -> cal err_pos_i agent 5/1(delta_ksi_vec)
  [delta_eta_vec] -> cal err_vel_i agent 1/1(delta_eta_vec)
  [delta_eta_vec] -> cal err_vel_i agent 2/1(delta_eta_vec)
  [delta_eta_vec] -> cal err_vel_i agent 3/1(delta_eta_vec)
  [delta_eta_vec] -> cal err_vel_i agent 4/1(delta_eta_vec)
  [delta_eta_vec] -> cal err_vel_i agent 5/1(delta_eta_vec)
  [dp_2] -> combine translational disturbance/2(dp_2)
  Constant286/1 -> generate translational disturbance agent 2/3(dp_phi_t)
  Constant293/1 -> generate translational disturbance agent 4/2(dp_ff_t)
  generate translational disturbance agent 5/1(dp_5) -> [dp_5]
  Constant297/1 -> generate translational disturbance agent 5/1(dp_aa_t)
  generate translational disturbance agent 1/1(dp_1) -> [dp_1]
  Constant292/1 -> generate translational disturbance agent 4/3(dp_phi_t)
  Constant288/1 -> generate translational disturbance agent 2/1(dp_aa_t)
  Constant290/1 -> generate translational disturbance agent 3/2(dp_ff_t)
  Constant285/1 -> generate translational disturbance agent 1/1(dp_aa_t)
  [tsim] -> generate translational disturbance agent 4/4(t)
  [tsim] -> generate translational disturbance agent 1/4(t)
  [dp_5] -> combine translational disturbance/5(dp_5)
  [dp_1] -> combine translational disturbance/1(dp_1)
  combine translational disturbance/1(dp_vec) -> [dp_vec]
  Constant295/1 -> generate translational disturbance agent 5/3(dp_phi_t)
  Constant296/1 -> generate translational disturbance agent 5/2(dp_ff_t)
  [tsim] -> generate translational disturbance agent 3/4(t)
  generate translational disturbance agent 2/1(dp_2) -> [dp_2]
  [dp_4] -> combine translational disturbance/4(dp_4)
  [tsim] -> generate translational disturbance agent 5/4(t)
  generate translational disturbance agent 3/1(dp_3) -> [dp_3]
  Constant294/1 -> generate translational disturbance agent 4/1(dp_aa_t)
  Constant244/1 -> generate translational disturbance agent 1/2(dp_ff_t)
  generate translational disturbance agent 4/1(dp_4) -> [dp_4]
  Constant289/1 -> generate translational disturbance agent 3/3(dp_phi_t)
  [dp_3] -> combine translational disturbance/3(dp_3)
  [tsim] -> generate translational disturbance agent 2/4(t)
  Constant243/1 -> generate translational disturbance agent 1/3(dp_phi_t)
  Constant291/1 -> generate translational disturbance agent 3/1(dp_aa_t)
  Constant287/1 -> generate translational disturbance agent 2/2(dp_ff_t)
  [delta_eta_vec] -> follower tracking error agent 1/2(delta_eta_vec)
  [delta_ksi_vec] -> follower tracking error agent 1/1(delta_ksi_vec)
  [delta_ksi_vec] -> follower tracking error agent 2/1(delta_ksi_vec)
  [delta_eta_vec] -> follower tracking error agent 2/2(delta_eta_vec)
  [delta_ksi_vec] -> follower tracking error agent 3/1(delta_ksi_vec)
  [delta_eta_vec] -> follower tracking error agent 3/2(delta_eta_vec)
  [delta_eta_vec] -> follower tracking error agent 4/2(delta_eta_vec)
  [delta_ksi_vec] -> follower tracking error agent 4/1(delta_ksi_vec)
  [delta_eta_vec] -> follower tracking error agent 5/2(delta_eta_vec)
  [delta_ksi_vec] -> follower tracking error agent 5/1(delta_ksi_vec)
  [delta_ksi_vec] -> cal Di agent 1/2(delta_ksi_vec)
  [delta_ksi_vec] -> cal Di agent 2/2(delta_ksi_vec)
  [delta_ksi_vec] -> cal Di agent 3/2(delta_ksi_vec)
  [delta_ksi_vec] -> cal Di agent 4/2(delta_ksi_vec)
  [delta_ksi_vec] -> cal Di agent 5/2(delta_ksi_vec)
  [delta_ksi_vec] -> To Workspace35/1
  [delta_eta_vec] -> To Workspace36/1
  [eta_est_err] -> To Workspace40/1
  [ksi_d_est_vec] -> To Workspace39/1
  [eta_d_est_vec] -> To Workspace37/1
  [ksi_est_err] -> To Workspace38/1
  [ksi_est_err_tilt_vec] -> choose eta_est_err_tilt 13/1(x)
  cal abs 53/1(y) -> Mux129/1
  Mux95/1 -> eta_d_est_2/1
  Mux93/1 -> eta_d_est_1/2
  Constant253/1 -> Mux110/3
  Add6/1 -> Demux93/1
  cal theta_ksi_est_err_tilt agent 1/1(theta_ksi_est_err_tilt_1_1) -> [theta_ksi_est_err_tilt_1_1]
  Demux72/2 -> Mux96/2
  Demux69/2 -> Mux93/1
  Demux92/3 -> Mux132/1
  Constant210/1 -> fixed-time distributed follower desire velocity observer agent 4/1(l1v)
  Demux88/1 -> Mux86/2
  Interpreted MATLAB Function55/1 -> trans to column55/1(x)
  [theta_ksi_est_err_tilt_2_vec] -> fixed-time distributed follower desire position observer agent 4/5(theta_ksi_est_err_tilt_2_vec)
  trans to column54/1(y) -> [eta_est_err_squ_1_node_1], Display93/1
  cal abs 60/1(y) -> Mux118/1
  velocity observe Integrator 4/1 -> [eta_d_est_4], Demux75/1
  [ksi_est_err_squ_1_node_1] -> cal theta_ksi_est_err_tilt agent 1/2(ksi_est_err_squ_1_node_1)
  Constant220/1 -> Mux122/2
  [ksi_d_est_5] -> combine leader position estimaters/5(ksi_d_est_5)
  fixed-time distributed follower desire position observer agent 5/1(d_ksi_d_est_5) -> position observe Integrator 5/1
  [theta_eta_est_err_tilt_1_4] -> combine lumped follower velocity observation error/4(theta_eta_est_err_tilt_1_4)
  trans to column47/1(y) -> [ksi_est_err_squ_1_node_3], Display81/1
  [theta_ksi_est_err_tilt_1_vec] -> fixed-time distributed follower desire position observer agent 3/4(theta_ksi_est_err_tilt_1_vec)
  Mux112/1 -> Interpreted MATLAB Function55/1
  Demux94/1 -> Mux133/1
  Constant246/1 -> Mux115/3
  Demux73/3 -> Mux101/1
  [eta_est_err_tilt_vec] -> choose eta_est_err_tilt 9/1(x)
  Demux75/2 -> Mux103/1
  [theta_eta_est_err_tilt_2_vec] -> fixed-time distributed follower desire velocity observer agent 2/4(theta_eta_est_err_tilt_2_vec)
  [ksi_est_err_tilt_vec] -> choose eta_est_err_tilt 14/1(x)
  Mux134/1 -> ksi_d_est_3/2
  Constant268/1 -> Mux121/2
  [ksi_d_est_2] -> combine leader position estimaters/2(ksi_d_est_2)
  trans to column46/1(y) -> [ksi_est_err_squ_2_node_3], Display80/1
  Demux93/2 -> Mux130/2
  fixed-time distributed follower desire position observer agent 1/1(d_ksi_d_est_1) -> position observe Integrator 1/1
  choose eta_est_err_tilt 11/1(y) -> cal abs 43/1(x)
  trans to column56/1(y) -> [eta_est_err_squ_1_node_3], Display90/1
  Mux133/1 -> ksi_d_est_3/1
  Constant230/1 -> fixed-time distributed follower desire position observer agent 2/1(l1p)
  Demux93/3 -> Mux132/2
  [theta_ksi_est_err_tilt_1_1] -> combine lumped follower position observation error/1(theta_ksi_est_err_tilt_1_1)
  cal abs 55/1(y) -> Mux110/1
  Demux92/2 -> Mux130/1
  Constant216/1 -> Mux126/3
  Mux99/1 -> eta_d_est_3/1
  Constant209/1 -> fixed-time distributed follower desire velocity observer agent 4/2(l2v)
  Interpreted MATLAB Function41/1 -> trans to column41/1(x)
  Mux120/1 -> Interpreted MATLAB Function42/1
  Mux115/1 -> Interpreted MATLAB Function54/1
  cal theta_ksi_est_err_tilt agent 3/1(theta_ksi_est_err_tilt_1_3) -> [theta_ksi_est_err_tilt_1_3]
  [ksi0] -> Add5/1
  [eta0] -> Add4/1
  fixed-time distributed follower desire position observer agent 4/1(d_ksi_d_est_4) -> position observe Integrator 4/1
  fixed-time distributed follower desire velocity observer agent 3/1(d_eta_d_est_3) -> velocity observe Integrator 3/1
  [theta_ksi_est_err_tilt_1_2] -> combine lumped follower position observation error/2(theta_ksi_est_err_tilt_1_2)
  Mux88/1 -> ksi_d_est_4/2
  choose eta_est_err_tilt 16/1(y) -> cal abs 48/1(x)
  [theta_eta_est_err_tilt_2_vec] -> fixed-time distributed follower desire velocity observer agent 4/4(theta_eta_est_err_tilt_2_vec)
  [eta_est_err_squ_2_node_4] -> cal theta_eta_est_err_tilt agent 4/3(eta_est_err_squ_2_node_4)
  cal theta_eta_est_err_tilt agent 4/1(theta_eta_est_err_tilt_1_4) -> [theta_eta_est_err_tilt_1_4]
  Constant133/1 -> fixed-time distributed follower desire position observer agent 1/1(l1p)
  Demux68/2 -> Mux91/1
  trans to column55/1(y) -> [eta_est_err_squ_2_node_3], Display89/1
  cal abs 56/1(y) -> Mux113/1
  Constant271/1 -> Mux124/3
  position observe Integrator 4/1 -> [ksi_d_est_4], Demux96/1
  Demux71/3 -> Mux98/1
  Interpreted MATLAB Function52/1 -> trans to column52/1(x)
  cal theta_eta_est_err_tilt agent 2/1(theta_eta_est_err_tilt_1_2) -> [theta_eta_est_err_tilt_1_2]
  cal abs 54/1(y) -> Mux111/1
  Constant264/1 -> Mux118/3
  Interpreted MATLAB Function56/1 -> trans to column56/1(x)
  Demux69/3 -> Mux94/1
  [eta0] -> Add3/1
  fixed-time distributed follower desire velocity observer agent 1/1(d_eta_d_est_1) -> velocity observe Integrator 1/1
  cal theta_ksi_est_err_tilt agent 3/2(theta_ksi_est_err_tilt_2_3) -> [theta_ksi_est_err_tilt_2_3]
  Constant202/1 -> fixed-time distributed follower desire velocity observer agent 2/2(l2v)
  cal theta_eta_est_err_tilt agent 1/2(theta_eta_est_err_tilt_2_1) -> [theta_eta_est_err_tilt_2_1]
  Constant251/1 -> Mux110/2
  cal abs 57/1(y) -> Mux112/1
  Mux124/1 -> Interpreted MATLAB Function47/1
  [eta_est_err_tilt_vec] -> choose eta_est_err_tilt 3/1(x)
  [theta_eta_est_err_tilt_1_5] -> combine lumped follower velocity observation error/5(theta_eta_est_err_tilt_1_5)
  [theta_eta_est_err_tilt_1_vec] -> fixed-time distributed follower desire velocity observer agent 1/3(theta_eta_est_err_tilt_1_vec)
  Constant260/1 -> Mux114/2
  Add9/1 -> Demux80/1
  Constant204/1 -> Add1/2
  choose eta_est_err_tilt 6/1(y) -> cal abs 57/1(x)
  Constant283/1 -> cal theta_ksi_est_err_tilt agent 1/1(alfa_theta)
  Mux96/1 -> eta_d_est_2/2
  Mux114/1 -> Interpreted MATLAB Function57/1
  [theta_ksi_est_err_tilt_2_1] -> combine lumped follower position observation error/6(theta_ksi_est_err_tilt_2_1)
  Mux98/1 -> eta_d_est_2/3
  Interpreted MATLAB Function49/1 -> trans to column49/1(x)
  [eta_d_est_vec] -> fixed-time distributed follower desire position observer agent 5/3(eta_d_est_vec)
  trans to column59/1(y) -> [eta_est_err_squ_2_node_5], Display94/1
  Demux95/3 -> Mux135/2
  Constant277/1 -> Mux125/2
  [theta_ksi_est_err_tilt_2_2] -> combine lumped follower position observation error/7(theta_ksi_est_err_tilt_2_2)
  [ksi_est_err_squ_1_node_4] -> cal theta_ksi_est_err_tilt agent 4/2(ksi_est_err_squ_1_node_4)
  Interpreted MATLAB Function59/1 -> trans to column59/1(x)
  [theta_eta_est_err_tilt_2_vec] -> fixed-time distributed follower desire velocity observer agent 1/4(theta_eta_est_err_tilt_2_vec)
  combine lumped follower velocity observation error/2(theta_eta_est_err_tilt_2_vec) -> [theta_eta_est_err_tilt_2_vec]
  Demux94/3 -> Mux135/1
  choose eta_est_err_tilt 19/1(y) -> cal abs 51/1(x)
  [eta_d_est_1] -> combine follower desire velocity estimaters/1(eta_d_est_1)
  [ksi_est_err_squ_1_node_2] -> cal theta_ksi_est_err_tilt agent 2/2(ksi_est_err_squ_1_node_2)
  cal abs 41/1(y) -> Mux115/1
  combine follower desire velocity estimaters/1(eta_d_est_vec) -> [eta_d_est_vec]
  [ksi_est_err_tilt_vec] -> choose eta_est_err_tilt 16/1(x)
  Demux70/1 -> Mux92/2
  [eta_d_est_vec] -> fixed-time distributed follower desire position observer agent 2/3(eta_d_est_vec)
  Constant219/1 -> fixed-time distributed follower desire position observer agent 2/2(l2p)
  velocity observe Integrator 3/1 -> [eta_d_est_3], Demux73/1
  Interpreted MATLAB Function57/1 -> trans to column57/1(x)
  cal theta_eta_est_err_tilt agent 5/2(theta_eta_est_err_tilt_2_5) -> [theta_eta_est_err_tilt_2_5]
  [theta_ksi_est_err_tilt_2_3] -> combine lumped follower position observation error/8(theta_ksi_est_err_tilt_2_3)
  Demux74/1 -> Mux99/2
  Constant200/1 -> fixed-time distributed follower desire velocity observer agent 1/1(l1v)
  Demux74/3 -> Mux101/2
  [eta0] -> Add/1
  Demux69/1 -> Mux92/1
  Demux79/3 -> Mux107/2
  [eta_d_est_vec] -> fixed-time distributed follower desire position observer agent 3/3(eta_d_est_vec)
  Mux116/1 -> Interpreted MATLAB Function58/1
  Constant252/1 -> fixed-time distributed follower desire position observer agent 3/2(l2p)
  fixed-time distributed follower desire position observer agent 2/1(d_ksi_d_est_2) -> position observe Integrator 2/1
  position observe Integrator 5/1 -> [ksi_d_est_5], Demux68/1
  [theta_ksi_est_err_tilt_2_vec] -> fixed-time distributed follower desire position observer agent 1/5(theta_ksi_est_err_tilt_2_vec)
  [eta_est_err_tilt_vec] -> choose eta_est_err_tilt 4/1(x)
  Mux100/1 -> eta_d_est_3/2
  choose eta_est_err_tilt 5/1(y) -> cal abs 56/1(x)
  cal abs 49/1(y) -> Mux123/1
  Constant245/1 -> Mux115/2
  [ksi_est_err_tilt_vec] -> choose eta_est_err_tilt 20/1(x)
  Mux103/1 -> eta_d_est_4/2
  choose eta_est_err_tilt 13/1(y) -> cal abs 45/1(x)
  Constant130/1 -> cal theta_eta_est_err_tilt agent 2/1(alfa_theta)
  Demux78/2 -> Mux97/1
  [theta_ksi_est_err_tilt_2_4] -> combine lumped follower position observation error/9(theta_ksi_est_err_tilt_2_4)
  [eta_est_err_tilt_vec] -> choose eta_est_err_tilt 2/1(x)
  [theta_eta_est_err_tilt_1_vec] -> fixed-time distributed follower desire velocity observer agent 2/3(theta_eta_est_err_tilt_1_vec)
  Demux95/1 -> Mux133/2
  Add1/1 -> Demux72/1
  Interpreted MATLAB Function44/1 -> trans to column44/1(x)
  Demux79/2 -> Mux106/2
  [theta_ksi_est_err_tilt_1_vec] -> fixed-time distributed follower desire position observer agent 2/4(theta_ksi_est_err_tilt_1_vec)
  [eta_est_err_squ_2_node_1] -> cal theta_eta_est_err_tilt agent 1/3(eta_est_err_squ_2_node_1)
  cal abs 47/1(y) -> Mux121/1
  choose eta_est_err_tilt 2/1(y) -> cal abs 52/1(x)
  [theta_eta_est_err_tilt_2_2] -> combine lumped follower velocity observation error/7(theta_eta_est_err_tilt_2_2)
  choose eta_est_err_tilt 4/1(y) -> cal abs 55/1(x)
  Constant213/1 -> fixed-time distributed follower desire velocity observer agent 5/1(l1v)
  Mux125/1 -> Interpreted MATLAB Function48/1
  trans to column41/1(y) -> [eta_est_err_squ_2_node_1], Display76/1
  [eta_d_est_vec] -> fixed-time distributed follower desire position observer agent 1/3(eta_d_est_vec)
  Constant64/1 -> Add8/2
  Interpreted MATLAB Function42/1 -> trans to column42/1(x)
  [eta_est_err_squ_2_node_3] -> cal theta_eta_est_err_tilt agent 3/3(eta_est_err_squ_2_node_3)
  Constant263/1 -> fixed-time distributed follower desire position observer agent 3/1(l1p)
  [eta_d_est_5] -> combine follower desire velocity estimaters/5(eta_d_est_5)
  [ksi_d_est_1] -> combine leader position estimaters/1(ksi_d_est_1)
  [eta_est_err_squ_1_node_5] -> cal theta_eta_est_err_tilt agent 5/2(eta_est_err_squ_1_node_5)
  Mux105/1 -> eta_d_est_5/1
  Constant207/1 -> Add2/2
  Demux88/2 -> Mux97/2
  Mux111/1 -> Interpreted MATLAB Function53/1
  choose eta_est_err_tilt 8/1(y) -> cal abs 59/1(x)
  Interpreted MATLAB Function51/1 -> trans to column51/1(x)
  Constant247/1 -> Mux109/2
  combine lumped follower position observation error/2(theta_ksi_est_err_tilt_2_vec) -> [theta_ksi_est_err_tilt_2_vec]
  Demux77/3 -> Mux107/1
  [eta_est_err_tilt_vec] -> choose eta_est_err_tilt 6/1(x)
  Constant45/1 -> fixed-time distributed follower desire position observer agent 1/2(l2p)
  [theta_ksi_est_err_tilt_1_5] -> combine lumped follower position observation error/5(theta_ksi_est_err_tilt_1_5)
  [eta_est_err_tilt_vec] -> choose eta_est_err_tilt 1/1(x)
  fixed-time distributed follower desire velocity observer agent 5/1(d_eta_d_est_5) -> velocity observe Integrator 5/1
  Constant262/1 -> Mux118/2
  Demux79/1 -> Mux105/2
  Constant208/1 -> Add5/2
  Mux130/1 -> ksi_d_est_2/2
  Interpreted MATLAB Function60/1 -> trans to column60/1(x)
  Constant254/1 -> Mux113/2
  Mux86/1 -> ksi_d_est_1/1
  position observe Integrator 1/1 -> [ksi_d_est_1], Demux78/1
  [eta0] -> Add2/1
  [ksi0] -> Add7/1
  Mux118/1 -> Interpreted MATLAB Function60/1
  Constant199/1 -> fixed-time distributed follower desire velocity observer agent 1/2(l2v)
  [theta_eta_est_err_tilt_2_vec] -> fixed-time distributed follower desire velocity observer agent 5/4(theta_eta_est_err_tilt_2_vec)
  [ksi0] -> Add9/1
  Mux129/1 -> Interpreted MATLAB Function51/1
  [eta_d_est_2] -> combine follower desire velocity estimaters/2(eta_d_est_2)
  Mux135/1 -> ksi_d_est_3/3
  Constant218/1 -> Mux120/3
  Demux71/2 -> Mux96/1
  Interpreted MATLAB Function47/1 -> trans to column47/1(x)
  trans to column52/1(y) -> [eta_est_err_squ_2_node_2], Display87/1
  Constant203/1 -> fixed-time distributed follower desire velocity observer agent 2/1(l1v)
  Constant131/1 -> cal theta_eta_est_err_tilt agent 3/1(alfa_theta)
  Constant250/1 -> Mux111/3
  choose eta_est_err_tilt 14/1(y) -> cal abs 46/1(x)
  cal theta_ksi_est_err_tilt agent 4/2(theta_ksi_est_err_tilt_2_4) -> [theta_ksi_est_err_tilt_2_4]
  Constant261/1 -> Mux114/3
  cal abs 59/1(y) -> Mux114/1
  [ksi_est_err_squ_1_node_3] -> cal theta_ksi_est_err_tilt agent 3/2(ksi_est_err_squ_1_node_3)
  velocity observe Integrator 2/1 -> [eta_d_est_2], Demux71/1
  [theta_eta_est_err_tilt_2_5] -> combine lumped follower velocity observation error/10(theta_eta_est_err_tilt_2_5)
  choose eta_est_err_tilt 1/1(y) -> cal abs 41/1(x)
  cal theta_eta_est_err_tilt agent 5/1(theta_eta_est_err_tilt_1_5) -> [theta_eta_est_err_tilt_1_5]
  cal theta_eta_est_err_tilt agent 3/2(theta_eta_est_err_tilt_2_3) -> [theta_eta_est_err_tilt_2_3]
  trans to column49/1(y) -> [ksi_est_err_squ_1_node_4], Display83/1
  Constant70/1 -> Add9/2
  fixed-time distributed follower desire velocity observer agent 2/1(d_eta_d_est_2) -> velocity observe Integrator 2/1
  Constant272/1 -> Mux123/2
  combine lumped follower position observation error/1(theta_ksi_est_err_tilt_1_vec) -> [theta_ksi_est_err_tilt_1_vec]
  Mux101/1 -> eta_d_est_3/3
  Mux92/1 -> eta_d_est_1/1
  Demux77/1 -> Mux105/1
  Demux68/3 -> Mux131/1
  cal abs 44/1(y) -> Mux128/1
  Demux96/1 -> Mux87/1
  Demux75/3 -> Mux104/1
  trans to column50/1(y) -> [ksi_est_err_squ_2_node_5], Display85/1
  cal theta_ksi_est_err_tilt agent 5/1(theta_ksi_est_err_tilt_1_5) -> [theta_ksi_est_err_tilt_1_5]
  trans to column42/1(y) -> [ksi_est_err_squ_2_node_1], Display77/1
  Interpreted MATLAB Function53/1 -> trans to column53/1(x)
  Constant46/1 -> fixed-time distributed follower desire position observer agent 4/2(l2p)
  Constant259/1 -> Mux116/3
  choose eta_est_err_tilt 18/1(y) -> cal abs 50/1(x)
  fixed-time distributed follower desire velocity observer agent 4/1(d_eta_d_est_4) -> velocity observe Integrator 4/1
  Constant201/1 -> Add/2
  Demux76/2 -> Mux103/2
  Demux75/1 -> Mux102/1
  Constant66/1 -> fixed-time distributed follower desire position observer agent 5/2(l2p)
  Constant205/1 -> fixed-time distributed follower desire velocity observer agent 3/2(l2v)
  Constant269/1 -> Mux121/3
  Demux70/2 -> Mux93/2
  [eta_est_err_tilt_vec] -> choose eta_est_err_tilt 10/1(x)
  [eta_est_err_tilt_vec] -> choose eta_est_err_tilt 5/1(x)
  Demux74/2 -> Mux100/2
  [ksi_est_err_tilt_vec] -> choose eta_est_err_tilt 18/1(x)
  [ksi_d_est_3] -> combine leader position estimaters/3(ksi_d_est_3)
  Demux73/1 -> Mux99/1
  Constant217/1 -> Mux120/2
  [ksi_est_err_squ_2_node_5] -> cal theta_ksi_est_err_tilt agent 5/3(ksi_est_err_squ_2_node_5)
  cal theta_eta_est_err_tilt agent 4/2(theta_eta_est_err_tilt_2_4) -> [theta_eta_est_err_tilt_2_4]
  [ksi_est_err_squ_2_node_1] -> cal theta_ksi_est_err_tilt agent 1/3(ksi_est_err_squ_2_node_1)
  Constant241/1 -> Add6/2
  Constant284/1 -> cal theta_ksi_est_err_tilt agent 2/1(alfa_theta)
  Mux132/1 -> ksi_d_est_2/3
  [eta_est_err_tilt_vec] -> cal theta_eta_est_err_tilt agent 4/4(eta_est_err_tilt_vec)
  Mux128/1 -> Interpreted MATLAB Function50/1
  Add7/1 -> Demux95/1
  Demux71/1 -> Mux95/1
  [theta_eta_est_err_tilt_2_vec] -> fixed-time distributed follower desire velocity observer agent 3/4(theta_eta_est_err_tilt_2_vec)
  trans to column57/1(y) -> [eta_est_err_squ_2_node_4], Display91/1
  Mux87/1 -> ksi_d_est_4/1
  Mux89/1 -> ksi_d_est_4/3
  Constant280/1 -> Mux129/3
  Demux68/1 -> Mux90/1
  Mux113/1 -> Interpreted MATLAB Function56/1
  [theta_eta_est_err_tilt_1_vec] -> fixed-time distributed follower desire velocity observer agent 5/3(theta_eta_est_err_tilt_1_vec)
  Demux88/3 -> Mux108/2
  [ksi_est_err_tilt_vec] -> choose eta_est_err_tilt 11/1(x)
  Constant48/1 -> cal theta_ksi_est_err_tilt agent 4/1(alfa_theta)
  [eta_d_est_3] -> combine follower desire velocity estimaters/3(eta_d_est_3)
  [theta_ksi_est_err_tilt_2_vec] -> fixed-time distributed follower desire position observer agent 3/5(theta_ksi_est_err_tilt_2_vec)
  [eta_est_err_squ_2_node_2] -> cal theta_eta_est_err_tilt agent 2/3(eta_est_err_squ_2_node_2)
  [theta_ksi_est_err_tilt_1_vec] -> fixed-time distributed follower desire position observer agent 1/4(theta_ksi_est_err_tilt_1_vec)
  [theta_eta_est_err_tilt_1_1] -> combine lumped follower velocity observation error/1(theta_eta_est_err_tilt_1_1)
  trans to column58/1(y) -> [eta_est_err_squ_1_node_4], Display92/1
  [theta_ksi_est_err_tilt_1_4] -> combine lumped follower position observation error/4(theta_ksi_est_err_tilt_1_4)
  [ksi_est_err_tilt_vec] -> cal theta_ksi_est_err_tilt agent 1/4(ksi_est_err_tilt_vec)
  Constant270/1 -> Mux124/2
  choose eta_est_err_tilt 20/1(y) -> cal abs 53/1(x)
  [theta_eta_est_err_tilt_2_4] -> combine lumped follower velocity observation error/9(theta_eta_est_err_tilt_2_4)
  Demux96/3 -> Mux89/1
  Constant198/1 -> cal theta_eta_est_err_tilt agent 5/1(alfa_theta)
  [eta_est_err_squ_1_node_1] -> cal theta_eta_est_err_tilt agent 1/2(eta_est_err_squ_1_node_1)
  [theta_eta_est_err_tilt_1_2] -> combine lumped follower velocity observation error/2(theta_eta_est_err_tilt_1_2)
  Demux80/1 -> Mux90/2
  Constant274/1 -> Add7/2
  Constant267/1 -> Mux122/3
  Mux108/1 -> ksi_d_est_1/3
  Demux80/3 -> Mux131/2
  Demux93/1 -> Mux119/2
  trans to column45/1(y) -> [ksi_est_err_squ_1_node_1], Display84/1
  Mux107/1 -> eta_d_est_5/3
  cal theta_ksi_est_err_tilt agent 2/2(theta_ksi_est_err_tilt_2_2) -> [theta_ksi_est_err_tilt_2_2]
  velocity observe Integrator 1/1 -> [eta_d_est_1], Demux69/1
  [theta_eta_est_err_tilt_1_vec] -> fixed-time distributed follower desire velocity observer agent 4/3(theta_eta_est_err_tilt_1_vec)
  choose eta_est_err_tilt 15/1(y) -> cal abs 47/1(x)
  Constant47/1 -> cal theta_ksi_est_err_tilt agent 3/1(alfa_theta)
  Constant62/1 -> fixed-time distributed follower desire position observer agent 4/1(l1p)
  [ksi_est_err_tilt_vec] -> choose eta_est_err_tilt 12/1(x)
  [eta_est_err_tilt_vec] -> choose eta_est_err_tilt 8/1(x)
  Demux94/2 -> Mux134/1
  Constant248/1 -> Mux109/3
  Demux78/1 -> Mux86/1
  cal theta_ksi_est_err_tilt agent 4/1(theta_ksi_est_err_tilt_1_4) -> [theta_ksi_est_err_tilt_1_4]
  Constant265/1 -> Mux117/2
  Constant132/1 -> cal theta_eta_est_err_tilt agent 4/1(alfa_theta)
  cal abs 58/1(y) -> Mux116/1
  Constant212/1 -> fixed-time distributed follower desire velocity observer agent 5/2(l2v)
  [eta_est_err_tilt_vec] -> cal theta_eta_est_err_tilt agent 3/4(eta_est_err_tilt_vec)
  Constant266/1 -> Mux117/3
  combine lumped follower velocity observation error/1(theta_eta_est_err_tilt_1_vec) -> [theta_eta_est_err_tilt_1_vec]
  choose eta_est_err_tilt 17/1(y) -> cal abs 49/1(x)
  cal theta_ksi_est_err_tilt agent 2/1(theta_ksi_est_err_tilt_1_2) -> [theta_ksi_est_err_tilt_1_2]
  Add5/1 -> Demux88/1
  Constant257/1 -> Mux112/3
  cal abs 42/1(y) -> Mux117/1
  trans to column51/1(y) -> [ksi_est_err_squ_1_node_5], Display86/1
  [theta_ksi_est_err_tilt_2_vec] -> fixed-time distributed follower desire position observer agent 2/5(theta_ksi_est_err_tilt_2_vec)
  Add/1 -> Demux70/1
  Demux97/1 -> Mux87/2
  Demux97/3 -> Mux89/2
  Mux94/1 -> eta_d_est_1/3
  [ksi_est_err_tilt_vec] -> cal theta_ksi_est_err_tilt agent 4/4(ksi_est_err_tilt_vec)
  Interpreted MATLAB Function48/1 -> trans to column48/1(x)
  Constant68/1 -> fixed-time distributed follower desire position observer agent 5/1(l1p)
  cal abs 43/1(y) -> Mux126/1
  Interpreted MATLAB Function45/1 -> trans to column45/1(x)
  Constant279/1 -> Mux129/2
  Add8/1 -> Demux97/1
  Interpreted MATLAB Function58/1 -> trans to column58/1(x)
  [ksi_est_err_squ_2_node_3] -> cal theta_ksi_est_err_tilt agent 3/3(ksi_est_err_squ_2_node_3)
  [ksi0] -> Add8/1
  Constant275/1 -> Mux127/2
  [eta_est_err_tilt_vec] -> cal theta_eta_est_err_tilt agent 1/4(eta_est_err_tilt_vec)
  Mux131/1 -> ksi_d_est_5/3
  [theta_ksi_est_err_tilt_2_5] -> combine lumped follower position observation error/10(theta_ksi_est_err_tilt_2_5)
  Add2/1 -> Demux74/1
  cal abs 52/1(y) -> Mux109/1
  [eta_d_est_vec] -> fixed-time distributed follower desire position observer agent 4/3(eta_d_est_vec)
  [theta_eta_est_err_tilt_1_3] -> combine lumped follower velocity observation error/3(theta_eta_est_err_tilt_1_3)
  Demux70/3 -> Mux94/2
  cal abs 45/1(y) -> Mux120/1
  Mux119/1 -> ksi_d_est_2/1
  Demux95/2 -> Mux134/2
  Mux102/1 -> eta_d_est_4/1
  combine leader position estimaters/1(ksi_d_est_vec) -> [ksi_d_est_vec]
  [eta_d_est_4] -> combine follower desire velocity estimaters/4(eta_d_est_4)
  Demux78/3 -> Mux108/1
  choose eta_est_err_tilt 7/1(y) -> cal abs 58/1(x)
  Mux127/1 -> Interpreted MATLAB Function49/1
  [eta_est_err_squ_1_node_3] -> cal theta_eta_est_err_tilt agent 3/2(eta_est_err_squ_1_node_3)
  Constant49/1 -> cal theta_ksi_est_err_tilt agent 5/1(alfa_theta)
  [theta_eta_est_err_tilt_2_1] -> combine lumped follower velocity observation error/6(theta_eta_est_err_tilt_2_1)
  [ksi_est_err_tilt_vec] -> choose eta_est_err_tilt 19/1(x)
  choose eta_est_err_tilt 3/1(y) -> cal abs 54/1(x)
  trans to column48/1(y) -> [ksi_est_err_squ_2_node_4], Display82/1
  [ksi_est_err_tilt_vec] -> cal theta_ksi_est_err_tilt agent 5/4(ksi_est_err_tilt_vec)
  Mux121/1 -> Interpreted MATLAB Function43/1
  cal theta_ksi_est_err_tilt agent 1/2(theta_ksi_est_err_tilt_2_1) -> [theta_ksi_est_err_tilt_2_1]
  position observe Integrator 2/1 -> [ksi_d_est_2], Demux92/1
  Mux123/1 -> Interpreted MATLAB Function46/1
  cal abs 46/1(y) -> Mux122/1
  [theta_ksi_est_err_tilt_1_3] -> combine lumped follower position observation error/3(theta_ksi_est_err_tilt_1_3)
  cal theta_eta_est_err_tilt agent 1/1(theta_eta_est_err_tilt_1_1) -> [theta_eta_est_err_tilt_1_1]
  Demux72/1 -> Mux95/2
  Constant129/1 -> cal theta_eta_est_err_tilt agent 1/1(alfa_theta)
  Demux73/2 -> Mux100/1
  Mux117/1 -> Interpreted MATLAB Function59/1
  Add4/1 -> Demux79/1
  cal abs 50/1(y) -> Mux127/1
  [eta_est_err_tilt_vec] -> cal theta_eta_est_err_tilt agent 5/4(eta_est_err_tilt_vec)
  Demux76/3 -> Mux104/2
  [eta_est_err_tilt_vec] -> choose eta_est_err_tilt 7/1(x)
  Constant282/1 -> Mux128/3
  [ksi_d_est_4] -> combine leader position estimaters/4(ksi_d_est_4)
  [ksi_est_err_squ_2_node_4] -> cal theta_ksi_est_err_tilt agent 4/3(ksi_est_err_squ_2_node_4)
  cal abs 51/1(y) -> Mux125/1
  [ksi_est_err_squ_2_node_2] -> cal theta_ksi_est_err_tilt agent 2/3(ksi_est_err_squ_2_node_2)
  Mux122/1 -> Interpreted MATLAB Function44/1
  Mux90/1 -> ksi_d_est_5/1
  Demux77/2 -> Mux106/1
  [eta_est_err_tilt_vec] -> cal theta_eta_est_err_tilt agent 2/4(eta_est_err_tilt_vec)
  cal theta_eta_est_err_tilt agent 3/1(theta_eta_est_err_tilt_1_3) -> [theta_eta_est_err_tilt_1_3]
  Mux97/1 -> ksi_d_est_1/2
  [theta_ksi_est_err_tilt_1_vec] -> fixed-time distributed follower desire position observer agent 4/4(theta_ksi_est_err_tilt_1_vec)
  choose eta_est_err_tilt 10/1(y) -> cal abs 42/1(x)
  Demux72/3 -> Mux98/2
  choose eta_est_err_tilt 9/1(y) -> cal abs 60/1(x)
  [ksi_est_err_tilt_vec] -> choose eta_est_err_tilt 15/1(x)
  [theta_ksi_est_err_tilt_1_vec] -> fixed-time distributed follower desire position observer agent 5/4(theta_ksi_est_err_tilt_1_vec)
  Mux106/1 -> eta_d_est_5/2
  Demux76/1 -> Mux102/2
  Constant211/1 -> Add3/2
  [eta0] -> Add1/1
  cal theta_ksi_est_err_tilt agent 5/2(theta_ksi_est_err_tilt_2_5) -> [theta_ksi_est_err_tilt_2_5]
  Mux110/1 -> Interpreted MATLAB Function52/1
  Constant255/1 -> Mux113/3
  [theta_eta_est_err_tilt_2_3] -> combine lumped follower velocity observation error/8(theta_eta_est_err_tilt_2_3)
  velocity observe Integrator 5/1 -> [eta_d_est_5], Demux77/1
  position observe Integrator 3/1 -> [ksi_d_est_3], Demux94/1
  Interpreted MATLAB Function54/1 -> trans to column54/1(x)
  trans to column60/1(y) -> [eta_est_err_squ_1_node_5], Display95/1
  Demux92/1 -> Mux119/1
  [eta_est_err_squ_1_node_2] -> cal theta_eta_est_err_tilt agent 2/2(eta_est_err_squ_1_node_2)
  [theta_eta_est_err_tilt_1_vec] -> fixed-time distributed follower desire velocity observer agent 3/3(theta_eta_est_err_tilt_1_vec)
  Interpreted MATLAB Function43/1 -> trans to column43/1(x)
  [ksi_est_err_tilt_vec] -> cal theta_ksi_est_err_tilt agent 2/4(ksi_est_err_tilt_vec)
  [eta_est_err_squ_1_node_4] -> cal theta_eta_est_err_tilt agent 4/2(eta_est_err_squ_1_node_4)
  choose eta_est_err_tilt 12/1(y) -> cal abs 44/1(x)
  Demux97/2 -> Mux88/2
  Constant214/1 -> Add4/2
  [ksi_est_err_tilt_vec] -> cal theta_ksi_est_err_tilt agent 3/4(ksi_est_err_tilt_vec)
  Constant278/1 -> Mux125/3
  [ksi0] -> Add6/1
  Constant249/1 -> Mux111/2
  Constant281/1 -> Mux128/2
  trans to column53/1(y) -> [eta_est_err_squ_1_node_2], Display88/1
  cal abs 48/1(y) -> Mux124/1
  Constant276/1 -> Mux127/3
  Mux104/1 -> eta_d_est_4/3
  [eta_est_err_squ_2_node_5] -> cal theta_eta_est_err_tilt agent 5/3(eta_est_err_squ_2_node_5)
  Interpreted MATLAB Function46/1 -> trans to column46/1(x)
  Interpreted MATLAB Function50/1 -> trans to column50/1(x)
  fixed-time distributed follower desire position observer agent 3/1(d_ksi_d_est_3) -> position observe Integrator 3/1
  Mux109/1 -> Interpreted MATLAB Function41/1
  Add3/1 -> Demux76/1
  Constant258/1 -> Mux116/2
  Constant215/1 -> Mux126/2
  Constant206/1 -> fixed-time distributed follower desire velocity observer agent 3/1(l1v)
  Demux80/2 -> Mux91/2
  [theta_ksi_est_err_tilt_2_vec] -> fixed-time distributed follower desire position observer agent 5/5(theta_ksi_est_err_tilt_2_vec)
  Demux96/2 -> Mux88/1
  trans to column44/1(y) -> [ksi_est_err_squ_1_node_2], Display79/1
  Constant273/1 -> Mux123/3
  Mux91/1 -> ksi_d_est_5/2
  Mux126/1 -> Interpreted MATLAB Function45/1
  [ksi_est_err_squ_1_node_5] -> cal theta_ksi_est_err_tilt agent 5/2(ksi_est_err_squ_1_node_5)
  trans to column43/1(y) -> [ksi_est_err_squ_2_node_2], Display78/1
  [ksi_est_err_tilt_vec] -> choose eta_est_err_tilt 17/1(x)
  cal theta_eta_est_err_tilt agent 2/2(theta_eta_est_err_tilt_2_2) -> [theta_eta_est_err_tilt_2_2]
  Constant256/1 -> Mux112/2
  [ksi0] -> cal lumped observation error agent 5/4(ksi0)
  cal lumped observation error agent 3/2(eta_est_err_tilt_3) -> [eta_est_err_tilt_3]
  Constant228/1 -> cal lumped observation error agent 2/2(w0)
  [eta0] -> cal lumped observation error agent 1/7(eta0)
  [eta0] -> cal lumped observation error agent 3/7(eta0)
  [eta_est_err_tilt_1] -> "combine lumped follower observation error "/6(eta_est_err_tilt_1)
  [eta_est_err_tilt_5] -> "combine lumped follower observation error "/10(eta_est_err_tilt_5)
  Constant240/1 -> cal lumped observation error agent 5/1(wij)
  [eta_d_est_vec] -> cal lumped observation error agent 5/6(eta_d_est_vec)
  [eta_est_err_tilt_2] -> "combine lumped follower observation error "/7(eta_est_err_tilt_2)
  [delta_ksi_vec] -> cal lumped observation error agent 3/5(delta_ksi_vec)
  cal lumped observation error agent 4/2(eta_est_err_tilt_4) -> [eta_est_err_tilt_4]
  [ksi_est_err_tilt_3] -> "combine lumped follower observation error "/3(ksi_est_err_tilt_3)
  [ksi_est_err_tilt_2] -> "combine lumped follower observation error "/2(ksi_est_err_tilt_2)
  [ksi_est_err_tilt_4] -> "combine lumped follower observation error "/4(ksi_est_err_tilt_4)
  [delta_eta_vec] -> cal lumped observation error agent 2/8(delta_eta_vec)
  [ksi_est_err_tilt_1] -> "combine lumped follower observation error "/1(ksi_est_err_tilt_1)
  [delta_ksi_vec] -> cal lumped observation error agent 5/5(delta_ksi_vec)
  [ksi0] -> cal lumped observation error agent 3/4(ksi0)
  Constant232/1 -> cal lumped observation error agent 3/1(wij)
  cal lumped observation error agent 5/1(ksi_est_err_tilt_5) -> [ksi_est_err_tilt_5]
  [ksi_est_err_tilt_5] -> "combine lumped follower observation error "/5(ksi_est_err_tilt_5)
  [eta_d_est_vec] -> cal lumped observation error agent 2/6(eta_d_est_vec)
  [eta_est_err_tilt_3] -> "combine lumped follower observation error "/8(eta_est_err_tilt_3)
  [delta_eta_vec] -> cal lumped observation error agent 4/8(delta_eta_vec)
  [ksi_d_est_vec] -> cal lumped observation error agent 5/3(ksi_d_est_vec)
  [eta_d_est_vec] -> cal lumped observation error agent 4/6(eta_d_est_vec)
  [delta_eta_vec] -> cal follower desire velocity estimate error/3(delta_eta_vec)
  [eta0] -> cal follower desire velocity estimate error/2(eta0)
  [eta_d_est_vec] -> cal lumped observation error agent 1/6(eta_d_est_vec)
  [delta_ksi_vec] -> cal follower desire position estimate error/3(delta_ksi_vec)
  [eta0] -> cal lumped observation error agent 4/7(eta0)
  [ksi_d_est_vec] -> cal lumped observation error agent 1/3(ksi_d_est_vec)
  [delta_eta_vec] -> cal lumped observation error agent 3/8(delta_eta_vec)
  cal lumped observation error agent 1/1(ksi_est_err_tilt_1) -> [ksi_est_err_tilt_1]
  cal follower desire velocity estimate error/1(eta_est_err) -> [eta_est_err]
  [delta_ksi_vec] -> cal lumped observation error agent 2/5(delta_ksi_vec)
  cal follower desire position estimate error/1(ksi_est_err) -> [ksi_est_err]
  Constant224/1 -> cal lumped observation error agent 1/2(w0)
  [eta_d_est_vec] -> cal follower desire velocity estimate error/1(eta_d_est_vec)
  cal lumped observation error agent 3/1(ksi_est_err_tilt_3) -> [ksi_est_err_tilt_3]
  [ksi0] -> cal follower desire position estimate error/2(ksi0)
  "combine lumped follower observation error "/1(ksi_est_err_tilt_vec) -> [ksi_est_err_tilt_vec]
  [eta0] -> cal lumped observation error agent 2/7(eta0)
  [ksi_d_est_vec] -> cal follower desire position estimate error/1(ksi_d_est_vec)
  Constant236/1 -> cal lumped observation error agent 4/1(wij)
  [eta_d_est_vec] -> cal lumped observation error agent 3/6(eta_d_est_vec)
  [ksi_d_est_vec] -> cal lumped observation error agent 3/3(ksi_d_est_vec)
  Constant242/1 -> cal lumped observation error agent 5/2(w0)
  [delta_ksi_vec] -> cal lumped observation error agent 4/5(delta_ksi_vec)
  [ksi0] -> cal lumped observation error agent 2/4(ksi0)
  cal lumped observation error agent 2/2(eta_est_err_tilt_2) -> [eta_est_err_tilt_2]
  Constant233/1 -> cal lumped observation error agent 3/2(w0)
  cal lumped observation error agent 4/1(ksi_est_err_tilt_4) -> [ksi_est_err_tilt_4]
  "combine lumped follower observation error "/2(eta_est_err_tilt_vec) -> [eta_est_err_tilt_vec]
  Constant237/1 -> cal lumped observation error agent 4/2(w0)
  [ksi_d_est_vec] -> cal lumped observation error agent 2/3(ksi_d_est_vec)
  [eta0] -> cal lumped observation error agent 5/7(eta0)
  Constant227/1 -> cal lumped observation error agent 2/1(wij)
  [ksi0] -> cal lumped observation error agent 4/4(ksi0)
  cal lumped observation error agent 5/2(eta_est_err_tilt_5) -> [eta_est_err_tilt_5]
  cal lumped observation error agent 1/2(eta_est_err_tilt_1) -> [eta_est_err_tilt_1]
  [delta_eta_vec] -> cal lumped observation error agent 5/8(delta_eta_vec)
  [ksi0] -> cal lumped observation error agent 1/4(ksi0)
  [delta_ksi_vec] -> cal lumped observation error agent 1/5(delta_ksi_vec)
  cal lumped observation error agent 2/1(ksi_est_err_tilt_2) -> [ksi_est_err_tilt_2]
  [delta_eta_vec] -> cal lumped observation error agent 1/8(delta_eta_vec)
  [eta_est_err_tilt_4] -> "combine lumped follower observation error "/9(eta_est_err_tilt_4)
  Constant223/1 -> cal lumped observation error agent 1/1(wij)
  [ksi_d_est_vec] -> cal lumped observation error agent 4/3(ksi_d_est_vec)
  [eta_d_est_vec] -> cal leader velocity observation/1(eta_d_est_vec)
  [delta_eta_vec] -> cal leader velocity observation/2(delta_eta_vec)
  cal leader velocity observation/1(eta_ld_hat_vec) -> Memory3/1
  Memory3/1 -> [eta_ld_hat_vec]
  cal leader position observation/1(ksi_ld_hat_vec) -> Memory7/1
  [ksi_d_est_vec] -> cal leader position observation/1(ksi_d_est_vec)
  [delta_ksi_vec] -> cal leader position observation/2(delta_ksi_vec)
  [eta_ld_hat_vec] -> cal leader velocity estimate error/1(eta_ld_hat_vec)
  [eta0] -> cal leader velocity estimate error/2(eta0)
  cal leader velocity estimate error/1(eta_ld_est_err) -> [eta_ld_est_err]
  cal leader position estimate error/1(ksi_ld_est_err) -> [ksi_ld_est_err]
  [ksi0] -> cal leader position estimate error/2(ksi0)
  [ksi_ld_hat_vec] -> cal leader position estimate error/1(ksi_ld_hat_vec)
  [eta_ld_est_err] -> To Workspace41/1
  [ksi_ld_est_err] -> To Workspace42/1
